simulink model "VAS_LEVEL0_TASK1_TIME"  (Simulink 3.00)
libraries: mathlib x438, logiclib x192, paramlib x18, genlib x3, timelib x1
(part 1 of 2)

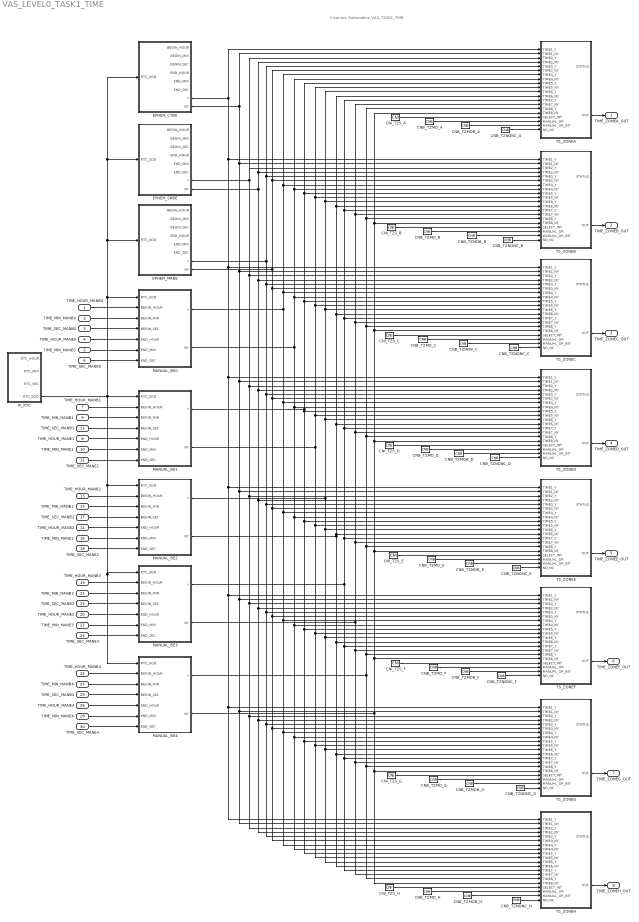
== system VAS_LEVEL0_TASK1_TIME ==
  note: Vivarium Automation VAS_TASK1_TIME
  TIME_HOUR_MANB0 : Inport  Port=1
  TIME_MIN_MANB0 : Inport  Port=2
  TIME_SEC_MANB0 : Inport  Port=3
  TIME_HOUR_MANE0 : Inport  Port=4
  TIME_MIN_MANE0 : Inport  Port=5
  TIME_SEC_MANE0 : Inport  Port=6
  TIME_HOUR_MANB1 : Inport  Port=7
  TIME_HOUR_MANE1 : Inport  Port=8
  TIME_MIN_MANB1 : Inport  Port=9
  TIME_MIN_MANE1 : Inport  Port=10
  TIME_SEC_MANB1 : Inport  Port=11
  TIME_SEC_MANE1 : Inport  Port=12
  TIME_HOUR_MANB2 : Inport  Port=13
  TIME_HOUR_MANE2 : Inport  Port=14
  TIME_MIN_MANB2 : Inport  Port=15
  TIME_MIN_MANE2 : Inport  Port=16
  TIME_SEC_MANB2 : Inport  Port=17
  TIME_SEC_MANE2 : Inport  Port=18
  TIME_HOUR_MANB3 : Inport  Port=19
  TIME_HOUR_MANE3 : Inport  Port=20
  TIME_MIN_MANB3 : Inport  Port=21
  TIME_MIN_MANE3 : Inport  Port=22
  TIME_SEC_MANB3 : Inport  Port=23
  TIME_SEC_MANE3 : Inport  Port=24
  TIME_HOUR_MANB4 : Inport  Port=25
  TIME_HOUR_MANE4 : Inport  Port=26
  TIME_MIN_MANB4 : Inport  Port=27
  TIME_MIN_MANE4 : Inport  Port=28
  TIME_SEC_MANB4 : Inport  Port=29
  TIME_SEC_MANE4 : Inport  Port=30
  CNB_TZMOB_A : mathlib/CNB  YCN=off
  CNB_TZMOB_B : mathlib/CNB  YCN=off
  CNB_TZMOB_C : mathlib/CNB  YCN=off
  CNB_TZMOB_D : mathlib/CNB  YCN=off
  CNB_TZMOB_E : mathlib/CNB  YCN=off
  CNB_TZMOB_F : mathlib/CNB  YCN=off
  CNB_TZMOB_G : mathlib/CNB  YCN=off
  CNB_TZMOB_H : mathlib/CNB  YCN=off
  CNB_TZMO_A : mathlib/CNB  YCN=off
  CNB_TZMO_B : mathlib/CNB  YCN=off
  CNB_TZMO_C : mathlib/CNB  YCN=off
  CNB_TZMO_D : mathlib/CNB  YCN=off
  CNB_TZMO_E : mathlib/CNB  YCN=off
  CNB_TZMO_F : mathlib/CNB  YCN=off
  CNB_TZMO_G : mathlib/CNB  YCN=off
  CNB_TZMO_H : mathlib/CNB  YCN=off
  CNB_TZNONC_A : mathlib/CNB  YCN=on
  CNB_TZNONC_B : mathlib/CNB  YCN=on
  CNB_TZNONC_C : mathlib/CNB  YCN=on
  CNB_TZNONC_D : mathlib/CNB  YCN=on
  CNB_TZNONC_E : mathlib/CNB  YCN=off
  CNB_TZNONC_F : mathlib/CNB  YCN=off
  CNB_TZNONC_G : mathlib/CNB  YCN=off
  CNB_TZNONC_H : mathlib/CNB  YCN=off
  CNI_TZS_A : mathlib/CNI  icn=0
  CNI_TZS_B : mathlib/CNI  icn=2
  CNI_TZS_C : mathlib/CNI  icn=1
  CNI_TZS_D : mathlib/CNI  icn=6
  CNI_TZS_E : mathlib/CNI  icn=16
  CNI_TZS_F : mathlib/CNI  icn=16
  CNI_TZS_G : mathlib/CNI  icn=16
  CNI_TZS_H : mathlib/CNI  icn=16
  EPHEM_CTBE : Subsystem
      mask Type: REX sequence
  EPHEM_MRBE : Subsystem
      mask Type: REX sequence
  EPHEM_SRBE : Subsystem
      mask Type: REX sequence
  MANUAL_BE0 : Subsystem
      mask Type: REX sequence
  MANUAL_BE1 : Subsystem
      mask Type: REX sequence
  MANUAL_BE2 : Subsystem
      mask Type: REX sequence
  MANUAL_BE3 : Subsystem
      mask Type: REX sequence
  MANUAL_BE4 : Subsystem
      mask Type: REX sequence
  PI_RTC : Subsystem
      mask Type: REX sequence
  TS_ZONEA : Subsystem
      mask Type: REX sequence
  TS_ZONEB : Subsystem
      mask Type: REX sequence
  TS_ZONEC : Subsystem
      mask Type: REX sequence
  TS_ZONED : Subsystem
      mask Type: REX sequence
  TS_ZONEE : Subsystem
      mask Type: REX sequence
  TS_ZONEF : Subsystem
      mask Type: REX sequence
  TS_ZONEG : Subsystem
      mask Type: REX sequence
  TS_ZONEH : Subsystem
      mask Type: REX sequence
  TIME_ZONEA_OUT : Outport  Port=1
  TIME_ZONEB_OUT : Outport  Port=2
  TIME_ZONEC_OUT : Outport  Port=3
  TIME_ZONED_OUT : Outport  Port=4
  TIME_ZONEE_OUT : Outport  Port=5
  TIME_ZONEF_OUT : Outport  Port=6
  TIME_ZONEG_OUT : Outport  Port=7
  TIME_ZONEH_OUT : Outport  Port=8
  wires:
  CNB_TZMOB_A/1 -> TS_ZONEA/19(MANUAL_OR_BIT)
  CNB_TZMOB_B/1 -> TS_ZONEB/19(MANUAL_OR_BIT)
  CNB_TZMOB_C/1 -> TS_ZONEC/19(MANUAL_OR_BIT)
  CNB_TZMOB_D/1 -> TS_ZONED/19(MANUAL_OR_BIT)
  CNB_TZMOB_E/1 -> TS_ZONEE/19(MANUAL_OR_BIT)
  CNB_TZMOB_F/1 -> TS_ZONEF/19(MANUAL_OR_BIT)
  CNB_TZMOB_G/1 -> TS_ZONEG/19(MANUAL_OR_BIT)
  CNB_TZMOB_H/1 -> TS_ZONEH/19(MANUAL_OR_BIT)
  CNB_TZMO_A/1 -> TS_ZONEA/18(MANUAL_OR)
  CNB_TZMO_B/1 -> TS_ZONEB/18(MANUAL_OR)
  CNB_TZMO_C/1 -> TS_ZONEC/18(MANUAL_OR)
  CNB_TZMO_D/1 -> TS_ZONED/18(MANUAL_OR)
  CNB_TZMO_E/1 -> TS_ZONEE/18(MANUAL_OR)
  CNB_TZMO_F/1 -> TS_ZONEF/18(MANUAL_OR)
  CNB_TZMO_G/1 -> TS_ZONEG/18(MANUAL_OR)
  CNB_TZMO_H/1 -> TS_ZONEH/18(MANUAL_OR)
  CNB_TZNONC_A/1 -> TS_ZONEA/20(NO_NC)
  CNB_TZNONC_B/1 -> TS_ZONEB/20(NO_NC)
  CNB_TZNONC_C/1 -> TS_ZONEC/20(NO_NC)
  CNB_TZNONC_D/1 -> TS_ZONED/20(NO_NC)
  CNB_TZNONC_E/1 -> TS_ZONEE/20(NO_NC)
  CNB_TZNONC_F/1 -> TS_ZONEF/20(NO_NC)
  CNB_TZNONC_G/1 -> TS_ZONEG/20(NO_NC)
  CNB_TZNONC_H/1 -> TS_ZONEH/20(NO_NC)
  CNI_TZS_A/1 -> TS_ZONEA/17(SELECT_INT)
  CNI_TZS_B/1 -> TS_ZONEB/17(SELECT_INT)
  CNI_TZS_C/1 -> TS_ZONEC/17(SELECT_INT)
  CNI_TZS_D/1 -> TS_ZONED/17(SELECT_INT)
  CNI_TZS_E/1 -> TS_ZONEE/17(SELECT_INT)
  CNI_TZS_F/1 -> TS_ZONEF/17(SELECT_INT)
  CNI_TZS_G/1 -> TS_ZONEG/17(SELECT_INT)
  CNI_TZS_H/1 -> TS_ZONEH/17(SELECT_INT)
  EPHEM_CTBE/7(Y) -> TS_ZONEA/1(TIME1_Y), TS_ZONEB/1(TIME1_Y), TS_ZONEC/1(TIME1_Y), TS_ZONED/1(TIME1_Y), TS_ZONEE/1(TIME1_Y), TS_ZONEG/1(TIME1_Y), TS_ZONEH/1(TIME1_Y), TS_ZONEF/1(TIME1_Y)
  EPHEM_CTBE/8(NY) -> TS_ZONEA/2(TIME1_NY), TS_ZONEB/2(TIME1_NY), TS_ZONEC/2(TIME1_NY), TS_ZONED/2(TIME1_NY), TS_ZONEE/2(TIME1_NY), TS_ZONEG/2(TIME1_NY), TS_ZONEH/2(TIME1_NY), TS_ZONEF/2(TIME1_NY)
  EPHEM_MRBE/7(Y) -> TS_ZONEA/5(TIME3_Y), TS_ZONEB/5(TIME3_Y), TS_ZONEC/5(TIME3_Y), TS_ZONED/5(TIME3_Y), TS_ZONEE/5(TIME3_Y), TS_ZONEG/5(TIME3_Y), TS_ZONEH/5(TIME3_Y), TS_ZONEF/5(TIME3_Y)
  EPHEM_MRBE/8(NY) -> TS_ZONEA/6(TIME3_NY), TS_ZONEB/6(TIME3_NY), TS_ZONEC/6(TIME3_NY), TS_ZONED/6(TIME3_NY), TS_ZONEE/6(TIME3_NY), TS_ZONEG/6(TIME3_NY), TS_ZONEH/6(TIME3_NY), TS_ZONEF/6(TIME3_NY)
  EPHEM_SRBE/7(Y) -> TS_ZONEC/3(TIME2_Y), TS_ZONED/3(TIME2_Y), TS_ZONEE/3(TIME2_Y), TS_ZONEG/3(TIME2_Y), TS_ZONEH/3(TIME2_Y), TS_ZONEF/3(TIME2_Y), TS_ZONEA/3(TIME2_Y), TS_ZONEB/3(TIME2_Y)
  EPHEM_SRBE/8(NY) -> TS_ZONEA/4(TIME2_NY), TS_ZONEB/4(TIME2_NY), TS_ZONEC/4(TIME2_NY), TS_ZONED/4(TIME2_NY), TS_ZONEE/4(TIME2_NY), TS_ZONEG/4(TIME2_NY), TS_ZONEH/4(TIME2_NY), TS_ZONEF/4(TIME2_NY)
  MANUAL_BE0/1(Y) -> TS_ZONEA/7(TIME4_Y), TS_ZONEB/7(TIME4_Y), TS_ZONEC/7(TIME4_Y), TS_ZONED/7(TIME4_Y), TS_ZONEE/7(TIME4_Y), TS_ZONEG/7(TIME4_Y), TS_ZONEH/7(TIME4_Y), TS_ZONEF/7(TIME4_Y)
  MANUAL_BE0/2(NY) -> TS_ZONEA/8(TIME4_NY), TS_ZONEB/8(TIME4_NY), TS_ZONEC/8(TIME4_NY), TS_ZONED/8(TIME4_NY), TS_ZONEE/8(TIME4_NY), TS_ZONEG/8(TIME4_NY), TS_ZONEH/8(TIME4_NY), TS_ZONEF/8(TIME4_NY)
  MANUAL_BE1/1(Y) -> TS_ZONEA/9(TIME5_Y), TS_ZONEB/9(TIME5_Y), TS_ZONEC/9(TIME5_Y), TS_ZONED/9(TIME5_Y), TS_ZONEE/9(TIME5_Y), TS_ZONEG/9(TIME5_Y), TS_ZONEH/9(TIME5_Y), TS_ZONEF/9(TIME5_Y)
  MANUAL_BE1/2(NY) -> TS_ZONEA/10(TIME5_NY), TS_ZONEB/10(TIME5_NY), TS_ZONEC/10(TIME5_NY), TS_ZONED/10(TIME5_NY), TS_ZONEE/10(TIME5_NY), TS_ZONEG/10(TIME5_NY), TS_ZONEH/10(TIME5_NY), TS_ZONEF/10(TIME5_NY)
  MANUAL_BE2/1(Y) -> TS_ZONEA/11(TIME6_Y), TS_ZONEB/11(TIME6_Y), TS_ZONEC/11(TIME6_Y), TS_ZONED/11(TIME6_Y), TS_ZONEE/11(TIME6_Y), TS_ZONEG/11(TIME6_Y), TS_ZONEH/11(TIME6_Y), TS_ZONEF/11(TIME6_Y)
  MANUAL_BE2/2(NY) -> TS_ZONEA/12(TIME6_NY), TS_ZONEB/12(TIME6_NY), TS_ZONEC/12(TIME6_NY), TS_ZONED/12(TIME6_NY), TS_ZONEE/12(TIME6_NY), TS_ZONEG/12(TIME6_NY), TS_ZONEH/12(TIME6_NY), TS_ZONEF/12(TIME6_NY)
  MANUAL_BE3/1(Y) -> TS_ZONEA/13(TIME7_Y), TS_ZONEB/13(TIME7_Y), TS_ZONEC/13(TIME7_Y), TS_ZONED/13(TIME7_Y), TS_ZONEE/13(TIME7_Y), TS_ZONEG/13(TIME7_Y), TS_ZONEH/13(TIME7_Y), TS_ZONEF/13(TIME7_Y)
  MANUAL_BE3/2(NY) -> TS_ZONEA/14(TIME7_NY), TS_ZONEB/14(TIME7_NY), TS_ZONEC/14(TIME7_NY), TS_ZONED/14(TIME7_NY), TS_ZONEE/14(TIME7_NY), TS_ZONEG/14(TIME7_NY), TS_ZONEH/14(TIME7_NY), TS_ZONEF/14(TIME7_NY)
  MANUAL_BE4/1(Y) -> TS_ZONEA/15(TIME8_Y), TS_ZONEB/15(TIME8_Y), TS_ZONEC/15(TIME8_Y), TS_ZONED/15(TIME8_Y), TS_ZONEE/15(TIME8_Y), TS_ZONEF/15(TIME8_Y), TS_ZONEG/15(TIME8_Y), TS_ZONEH/15(TIME8_Y)
  MANUAL_BE4/2(NY) -> TS_ZONEA/16(TIME8_NY), TS_ZONEB/16(TIME8_NY), TS_ZONEC/16(TIME8_NY), TS_ZONED/16(TIME8_NY), TS_ZONEE/16(TIME8_NY), TS_ZONEF/16(TIME8_NY), TS_ZONEG/16(TIME8_NY), TS_ZONEH/16(TIME8_NY)
  PI_RTC/4(RTC_SOD) -> MANUAL_BE3/1(RTC_SOD), MANUAL_BE4/1(RTC_SOD), MANUAL_BE2/1(RTC_SOD), EPHEM_CTBE/1(RTC_SOD), EPHEM_SRBE/1(RTC_SOD), EPHEM_MRBE/1(RTC_SOD), MANUAL_BE0/1(RTC_SOD), MANUAL_BE1/1(RTC_SOD)
  TIME_HOUR_MANB0/1 -> MANUAL_BE0/2(BEGIN_HOUR)
  TIME_HOUR_MANB1/1 -> MANUAL_BE1/2(BEGIN_HOUR)
  TIME_HOUR_MANB2/1 -> MANUAL_BE2/2(BEGIN_HOUR)
  TIME_HOUR_MANB3/1 -> MANUAL_BE3/2(BEGIN_HOUR)
  TIME_HOUR_MANB4/1 -> MANUAL_BE4/2(BEGIN_HOUR)
  TIME_HOUR_MANE0/1 -> MANUAL_BE0/5(END_HOUR)
  TIME_HOUR_MANE1/1 -> MANUAL_BE1/5(END_HOUR)
  TIME_HOUR_MANE2/1 -> MANUAL_BE2/5(END_HOUR)
  TIME_HOUR_MANE3/1 -> MANUAL_BE3/5(END_HOUR)
  TIME_HOUR_MANE4/1 -> MANUAL_BE4/5(END_HOUR)
  TIME_MIN_MANB0/1 -> MANUAL_BE0/3(BEGIN_MIN)
  TIME_MIN_MANB1/1 -> MANUAL_BE1/3(BEGIN_MIN)
  TIME_MIN_MANB2/1 -> MANUAL_BE2/3(BEGIN_MIN)
  TIME_MIN_MANB3/1 -> MANUAL_BE3/3(BEGIN_MIN)
  TIME_MIN_MANB4/1 -> MANUAL_BE4/3(BEGIN_MIN)
  TIME_MIN_MANE0/1 -> MANUAL_BE0/6(END_MIN)
  TIME_MIN_MANE1/1 -> MANUAL_BE1/6(END_MIN)
  TIME_MIN_MANE2/1 -> MANUAL_BE2/6(END_MIN)
  TIME_MIN_MANE3/1 -> MANUAL_BE3/6(END_MIN)
  TIME_MIN_MANE4/1 -> MANUAL_BE4/6(END_MIN)
  TIME_SEC_MANB0/1 -> MANUAL_BE0/4(BEGIN_SEC)
  TIME_SEC_MANB1/1 -> MANUAL_BE1/4(BEGIN_SEC)
  TIME_SEC_MANB2/1 -> MANUAL_BE2/4(BEGIN_SEC)
  TIME_SEC_MANB3/1 -> MANUAL_BE3/4(BEGIN_SEC)
  TIME_SEC_MANB4/1 -> MANUAL_BE4/4(BEGIN_SEC)
  TIME_SEC_MANE0/1 -> MANUAL_BE0/7(END_SEC)
  TIME_SEC_MANE1/1 -> MANUAL_BE1/7(END_SEC)
  TIME_SEC_MANE2/1 -> MANUAL_BE2/7(END_SEC)
  TIME_SEC_MANE3/1 -> MANUAL_BE3/7(END_SEC)
  TIME_SEC_MANE4/1 -> MANUAL_BE4/7(END_SEC)
  TS_ZONEA/2(OUT) -> TIME_ZONEA_OUT/1
  TS_ZONEB/2(OUT) -> TIME_ZONEB_OUT/1
  TS_ZONEC/2(OUT) -> TIME_ZONEC_OUT/1
  TS_ZONED/2(OUT) -> TIME_ZONED_OUT/1
  TS_ZONEE/2(OUT) -> TIME_ZONEE_OUT/1
  TS_ZONEF/2(OUT) -> TIME_ZONEF_OUT/1
  TS_ZONEG/2(OUT) -> TIME_ZONEG_OUT/1
  TS_ZONEH/2(OUT) -> TIME_ZONEH_OUT/1

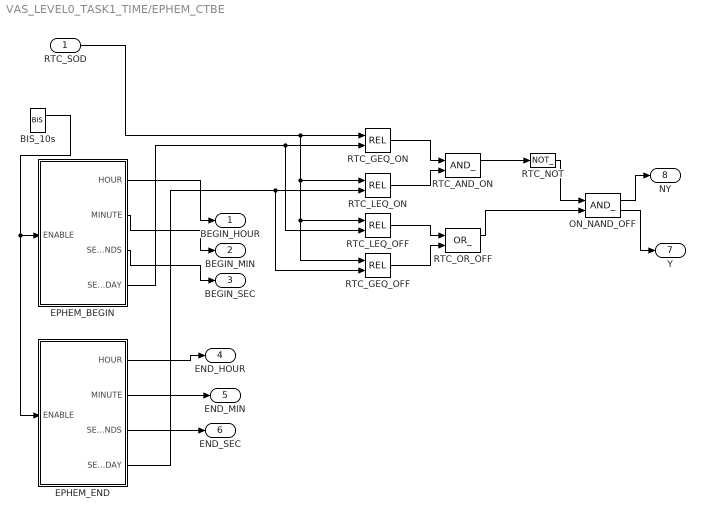
== system VAS_LEVEL0_TASK1_TIME/EPHEM_CTBE ==
  RTC_SOD : Inport  Port=1
  BIS_10s : genlib/BIS  Y0=off  t1=0  t2=1  t3=30  t4=4  t5=5  t6=6  t7=7  t8=8  RPT=on  bEdit=off
  EPHEM_BEGIN : Subsystem
      mask Type: REX sequence
  EPHEM_END : Subsystem
      mask Type: REX sequence
  ON_NAND_OFF : logiclib/AND_
  RTC_AND_ON : logiclib/AND_
  RTC_GEQ_OFF : mathlib/REL  irel=6: greater or equal (>=)
  RTC_GEQ_ON : mathlib/REL  irel=6: greater or equal (>=)
  RTC_LEQ_OFF : mathlib/REL  irel=5: less or equal (<=)
  RTC_LEQ_ON : mathlib/REL  irel=5: less or equal (<=)
  RTC_NOT : logiclib/NOT_
  RTC_OR_OFF : logiclib/OR_
  BEGIN_HOUR : Outport  Port=1
  BEGIN_MIN : Outport  Port=2
  BEGIN_SEC : Outport  Port=3
  END_HOUR : Outport  Port=4
  END_MIN : Outport  Port=5
  END_SEC : Outport  Port=6
  Y : Outport  Port=7
  NY : Outport  Port=8
  wires:
  BIS_10s/1 -> EPHEM_BEGIN/1(ENABLE), EPHEM_END/1(ENABLE)
  EPHEM_BEGIN/1(HOUR) -> BEGIN_HOUR/1
  EPHEM_BEGIN/2(MINUTE) -> BEGIN_MIN/1
  EPHEM_BEGIN/3(SECONDS) -> BEGIN_SEC/1
  EPHEM_BEGIN/4(SEC_OF_DAY) -> RTC_GEQ_ON/2, RTC_LEQ_OFF/2
  EPHEM_END/1(HOUR) -> END_HOUR/1
  EPHEM_END/2(MINUTE) -> END_MIN/1
  EPHEM_END/3(SECONDS) -> END_SEC/1
  EPHEM_END/4(SEC_OF_DAY) -> RTC_GEQ_OFF/2, RTC_LEQ_ON/2
  ON_NAND_OFF/1 -> NY/1
  ON_NAND_OFF/2 -> Y/1
  RTC_AND_ON/1 -> RTC_NOT/1
  RTC_GEQ_OFF/1 -> RTC_OR_OFF/2
  RTC_GEQ_ON/1 -> RTC_AND_ON/1
  RTC_LEQ_OFF/1 -> RTC_OR_OFF/1
  RTC_LEQ_ON/1 -> RTC_AND_ON/2
  RTC_NOT/1 -> ON_NAND_OFF/1
  RTC_OR_OFF/1 -> ON_NAND_OFF/2
  RTC_SOD/1 -> RTC_GEQ_ON/1, RTC_GEQ_OFF/1, RTC_LEQ_OFF/1, RTC_LEQ_ON/1

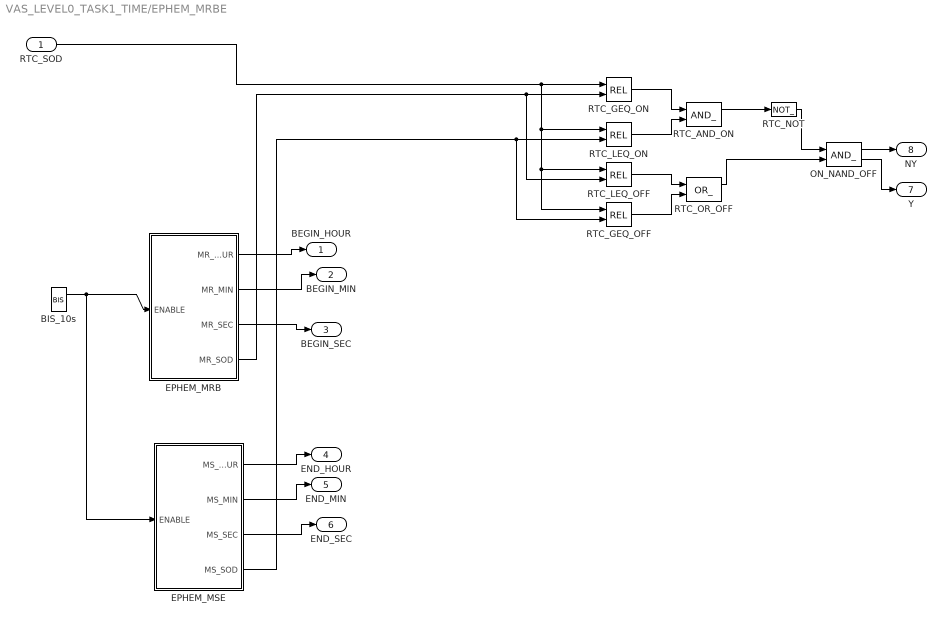
== system VAS_LEVEL0_TASK1_TIME/EPHEM_MRBE ==
  RTC_SOD : Inport  Port=1
  BIS_10s : genlib/BIS  Y0=off  t1=0  t2=1  t3=30  t4=4  t5=5  t6=6  t7=7  t8=8  RPT=on  bEdit=off
  EPHEM_MRB : Subsystem
      mask Type: REX sequence
  EPHEM_MSE : Subsystem
      mask Type: REX sequence
  ON_NAND_OFF : logiclib/AND_
  RTC_AND_ON : logiclib/AND_
  RTC_GEQ_OFF : mathlib/REL  irel=6: greater or equal (>=)
  RTC_GEQ_ON : mathlib/REL  irel=6: greater or equal (>=)
  RTC_LEQ_OFF : mathlib/REL  irel=5: less or equal (<=)
  RTC_LEQ_ON : mathlib/REL  irel=5: less or equal (<=)
  RTC_NOT : logiclib/NOT_
  RTC_OR_OFF : logiclib/OR_
  BEGIN_HOUR : Outport  Port=1
  BEGIN_MIN : Outport  Port=2
  BEGIN_SEC : Outport  Port=3
  END_HOUR : Outport  Port=4
  END_MIN : Outport  Port=5
  END_SEC : Outport  Port=6
  Y : Outport  Port=7
  NY : Outport  Port=8
  wires:
  BIS_10s/1 -> EPHEM_MRB/1(ENABLE), EPHEM_MSE/1(ENABLE)
  EPHEM_MRB/1(MR_HOUR) -> BEGIN_HOUR/1
  EPHEM_MRB/2(MR_MIN) -> BEGIN_MIN/1
  EPHEM_MRB/3(MR_SEC) -> BEGIN_SEC/1
  EPHEM_MRB/4(MR_SOD) -> RTC_GEQ_ON/2, RTC_LEQ_OFF/2
  EPHEM_MSE/1(MS_HOUR) -> END_HOUR/1
  EPHEM_MSE/2(MS_MIN) -> END_MIN/1
  EPHEM_MSE/3(MS_SEC) -> END_SEC/1
  EPHEM_MSE/4(MS_SOD) -> RTC_GEQ_OFF/2, RTC_LEQ_ON/2
  ON_NAND_OFF/1 -> NY/1
  ON_NAND_OFF/2 -> Y/1
  RTC_AND_ON/1 -> RTC_NOT/1
  RTC_GEQ_OFF/1 -> RTC_OR_OFF/2
  RTC_GEQ_ON/1 -> RTC_AND_ON/1
  RTC_LEQ_OFF/1 -> RTC_OR_OFF/1
  RTC_LEQ_ON/1 -> RTC_AND_ON/2
  RTC_NOT/1 -> ON_NAND_OFF/1
  RTC_OR_OFF/1 -> ON_NAND_OFF/2
  RTC_SOD/1 -> RTC_GEQ_ON/1, RTC_GEQ_OFF/1, RTC_LEQ_OFF/1, RTC_LEQ_ON/1

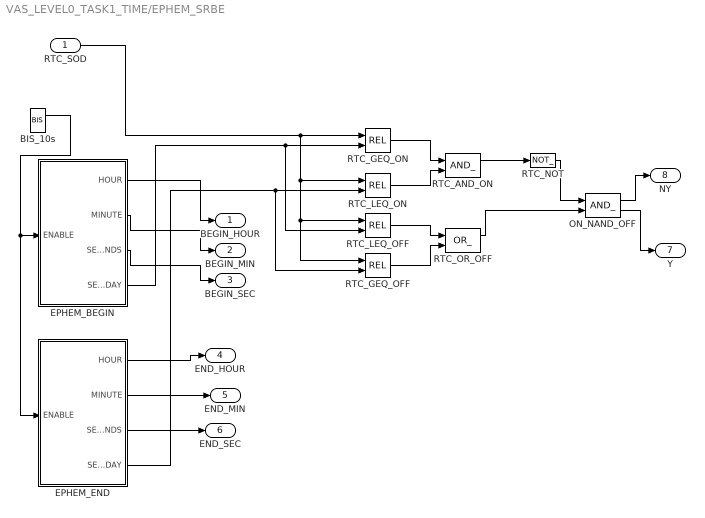
== system VAS_LEVEL0_TASK1_TIME/EPHEM_SRBE ==
  RTC_SOD : Inport  Port=1
  BIS_10s : genlib/BIS  Y0=off  t1=0  t2=1  t3=30  t4=4  t5=5  t6=6  t7=7  t8=8  RPT=on  bEdit=off
  EPHEM_BEGIN : Subsystem
      mask Type: REX sequence
  EPHEM_END : Subsystem
      mask Type: REX sequence
  ON_NAND_OFF : logiclib/AND_
  RTC_AND_ON : logiclib/AND_
  RTC_GEQ_OFF : mathlib/REL  irel=6: greater or equal (>=)
  RTC_GEQ_ON : mathlib/REL  irel=6: greater or equal (>=)
  RTC_LEQ_OFF : mathlib/REL  irel=5: less or equal (<=)
  RTC_LEQ_ON : mathlib/REL  irel=5: less or equal (<=)
  RTC_NOT : logiclib/NOT_
  RTC_OR_OFF : logiclib/OR_
  BEGIN_HOUR : Outport  Port=1
  BEGIN_MIN : Outport  Port=2
  BEGIN_SEC : Outport  Port=3
  END_HOUR : Outport  Port=4
  END_MIN : Outport  Port=5
  END_SEC : Outport  Port=6
  Y : Outport  Port=7
  NY : Outport  Port=8
  wires:
  BIS_10s/1 -> EPHEM_BEGIN/1(ENABLE), EPHEM_END/1(ENABLE)
  EPHEM_BEGIN/1(HOUR) -> BEGIN_HOUR/1
  EPHEM_BEGIN/2(MINUTE) -> BEGIN_MIN/1
  EPHEM_BEGIN/3(SECONDS) -> BEGIN_SEC/1
  EPHEM_BEGIN/4(SEC_OF_DAY) -> RTC_GEQ_ON/2, RTC_LEQ_OFF/2
  EPHEM_END/1(HOUR) -> END_HOUR/1
  EPHEM_END/2(MINUTE) -> END_MIN/1
  EPHEM_END/3(SECONDS) -> END_SEC/1
  EPHEM_END/4(SEC_OF_DAY) -> RTC_GEQ_OFF/2, RTC_LEQ_ON/2
  ON_NAND_OFF/1 -> NY/1
  ON_NAND_OFF/2 -> Y/1
  RTC_AND_ON/1 -> RTC_NOT/1
  RTC_GEQ_OFF/1 -> RTC_OR_OFF/2
  RTC_GEQ_ON/1 -> RTC_AND_ON/1
  RTC_LEQ_OFF/1 -> RTC_OR_OFF/1
  RTC_LEQ_ON/1 -> RTC_AND_ON/2
  RTC_NOT/1 -> ON_NAND_OFF/1
  RTC_OR_OFF/1 -> ON_NAND_OFF/2
  RTC_SOD/1 -> RTC_GEQ_ON/1, RTC_GEQ_OFF/1, RTC_LEQ_OFF/1, RTC_LEQ_ON/1

== system VAS_LEVEL0_TASK1_TIME/MANUAL_BE0 ==
  RTC_SOD : Inport  Port=1
  BEGIN_HOUR : Inport  Port=2
  BEGIN_MIN : Inport  Port=3
  BEGIN_SEC : Inport  Port=4
  END_HOUR : Inport  Port=5
  END_MIN : Inport  Port=6
  END_SEC : Inport  Port=7
  MANUAL_BEGIN : Subsystem
      mask Type: REX sequence
  MANUAL_END : Subsystem
      mask Type: REX sequence
  ON_NAND_OFF : logiclib/AND_
  RTC_AND_ON : logiclib/AND_
  RTC_GEQ_OFF : mathlib/REL  irel=6: greater or equal (>=)
  RTC_GEQ_ON : mathlib/REL  irel=6: greater or equal (>=)
  RTC_LEQ_OFF : mathlib/REL  irel=5: less or equal (<=)
  RTC_LEQ_ON : mathlib/REL  irel=5: less or equal (<=)
  RTC_NOT : logiclib/NOT_
  RTC_OR_OFF : logiclib/OR_
  Y : Outport  Port=1
  NY : Outport  Port=2
  wires:
  BEGIN_HOUR/1 -> MANUAL_BEGIN/1(IN_HOUR)
  BEGIN_MIN/1 -> MANUAL_BEGIN/2(IN_MINUTE)
  BEGIN_SEC/1 -> MANUAL_BEGIN/3(IN_SECONDS)
  END_HOUR/1 -> MANUAL_END/1(IN_HOUR)
  END_MIN/1 -> MANUAL_END/2(IN_MINUTE)
  END_SEC/1 -> MANUAL_END/3(IN_SECONDS)
  MANUAL_BEGIN/4(SEC_OF_DAY) -> RTC_GEQ_ON/2, RTC_LEQ_OFF/2
  MANUAL_END/4(SEC_OF_DAY) -> RTC_GEQ_OFF/2, RTC_LEQ_ON/2
  ON_NAND_OFF/1 -> NY/1
  ON_NAND_OFF/2 -> Y/1
  RTC_AND_ON/1 -> RTC_NOT/1
  RTC_GEQ_OFF/1 -> RTC_OR_OFF/2
  RTC_GEQ_ON/1 -> RTC_AND_ON/1
  RTC_LEQ_OFF/1 -> RTC_OR_OFF/1
  RTC_LEQ_ON/1 -> RTC_AND_ON/2
  RTC_NOT/1 -> ON_NAND_OFF/1
  RTC_OR_OFF/1 -> ON_NAND_OFF/2
  RTC_SOD/1 -> RTC_GEQ_ON/1, RTC_GEQ_OFF/1, RTC_LEQ_OFF/1, RTC_LEQ_ON/1

== system VAS_LEVEL0_TASK1_TIME/MANUAL_BE1 ==
  RTC_SOD : Inport  Port=1
  BEGIN_HOUR : Inport  Port=2
  BEGIN_MIN : Inport  Port=3
  BEGIN_SEC : Inport  Port=4
  END_HOUR : Inport  Port=5
  END_MIN : Inport  Port=6
  END_SEC : Inport  Port=7
  MANUAL_BEGIN : Subsystem
      mask Type: REX sequence
  MANUAL_END : Subsystem
      mask Type: REX sequence
  ON_NAND_OFF : logiclib/AND_
  RTC_AND_ON : logiclib/AND_
  RTC_GEQ_OFF : mathlib/REL  irel=6: greater or equal (>=)
  RTC_GEQ_ON : mathlib/REL  irel=6: greater or equal (>=)
  RTC_LEQ_OFF : mathlib/REL  irel=5: less or equal (<=)
  RTC_LEQ_ON : mathlib/REL  irel=5: less or equal (<=)
  RTC_NOT : logiclib/NOT_
  RTC_OR_OFF : logiclib/OR_
  Y : Outport  Port=1
  NY : Outport  Port=2
  wires:
  BEGIN_HOUR/1 -> MANUAL_BEGIN/1(IN_HOUR)
  BEGIN_MIN/1 -> MANUAL_BEGIN/2(IN_MINUTE)
  BEGIN_SEC/1 -> MANUAL_BEGIN/3(IN_SECONDS)
  END_HOUR/1 -> MANUAL_END/1(IN_HOUR)
  END_MIN/1 -> MANUAL_END/2(IN_MINUTE)
  END_SEC/1 -> MANUAL_END/3(IN_SECONDS)
  MANUAL_BEGIN/4(SEC_OF_DAY) -> RTC_GEQ_ON/2, RTC_LEQ_OFF/2
  MANUAL_END/4(SEC_OF_DAY) -> RTC_GEQ_OFF/2, RTC_LEQ_ON/2
  ON_NAND_OFF/1 -> NY/1
  ON_NAND_OFF/2 -> Y/1
  RTC_AND_ON/1 -> RTC_NOT/1
  RTC_GEQ_OFF/1 -> RTC_OR_OFF/2
  RTC_GEQ_ON/1 -> RTC_AND_ON/1
  RTC_LEQ_OFF/1 -> RTC_OR_OFF/1
  RTC_LEQ_ON/1 -> RTC_AND_ON/2
  RTC_NOT/1 -> ON_NAND_OFF/1
  RTC_OR_OFF/1 -> ON_NAND_OFF/2
  RTC_SOD/1 -> RTC_GEQ_ON/1, RTC_GEQ_OFF/1, RTC_LEQ_OFF/1, RTC_LEQ_ON/1

== system VAS_LEVEL0_TASK1_TIME/MANUAL_BE2 ==
  RTC_SOD : Inport  Port=1
  BEGIN_HOUR : Inport  Port=2
  BEGIN_MIN : Inport  Port=3
  BEGIN_SEC : Inport  Port=4
  END_HOUR : Inport  Port=5
  END_MIN : Inport  Port=6
  END_SEC : Inport  Port=7
  MANUAL_BEGIN : Subsystem
      mask Type: REX sequence
  MANUAL_END : Subsystem
      mask Type: REX sequence
  ON_NAND_OFF : logiclib/AND_
  RTC_AND_ON : logiclib/AND_
  RTC_GEQ_OFF : mathlib/REL  irel=6: greater or equal (>=)
  RTC_GEQ_ON : mathlib/REL  irel=6: greater or equal (>=)
  RTC_LEQ_OFF : mathlib/REL  irel=5: less or equal (<=)
  RTC_LEQ_ON : mathlib/REL  irel=5: less or equal (<=)
  RTC_NOT : logiclib/NOT_
  RTC_OR_OFF : logiclib/OR_
  Y : Outport  Port=1
  NY : Outport  Port=2
  wires:
  BEGIN_HOUR/1 -> MANUAL_BEGIN/1(IN_HOUR)
  BEGIN_MIN/1 -> MANUAL_BEGIN/2(IN_MINUTE)
  BEGIN_SEC/1 -> MANUAL_BEGIN/3(IN_SECONDS)
  END_HOUR/1 -> MANUAL_END/1(IN_HOUR)
  END_MIN/1 -> MANUAL_END/2(IN_MINUTE)
  END_SEC/1 -> MANUAL_END/3(IN_SECONDS)
  MANUAL_BEGIN/4(SEC_OF_DAY) -> RTC_GEQ_ON/2, RTC_LEQ_OFF/2
  MANUAL_END/4(SEC_OF_DAY) -> RTC_GEQ_OFF/2, RTC_LEQ_ON/2
  ON_NAND_OFF/1 -> NY/1
  ON_NAND_OFF/2 -> Y/1
  RTC_AND_ON/1 -> RTC_NOT/1
  RTC_GEQ_OFF/1 -> RTC_OR_OFF/2
  RTC_GEQ_ON/1 -> RTC_AND_ON/1
  RTC_LEQ_OFF/1 -> RTC_OR_OFF/1
  RTC_LEQ_ON/1 -> RTC_AND_ON/2
  RTC_NOT/1 -> ON_NAND_OFF/1
  RTC_OR_OFF/1 -> ON_NAND_OFF/2
  RTC_SOD/1 -> RTC_GEQ_ON/1, RTC_GEQ_OFF/1, RTC_LEQ_OFF/1, RTC_LEQ_ON/1

== system VAS_LEVEL0_TASK1_TIME/MANUAL_BE3 ==
  RTC_SOD : Inport  Port=1
  BEGIN_HOUR : Inport  Port=2
  BEGIN_MIN : Inport  Port=3
  BEGIN_SEC : Inport  Port=4
  END_HOUR : Inport  Port=5
  END_MIN : Inport  Port=6
  END_SEC : Inport  Port=7
  MANUAL_BEGIN : Subsystem
      mask Type: REX sequence
  MANUAL_END : Subsystem
      mask Type: REX sequence
  ON_NAND_OFF : logiclib/AND_
  RTC_AND_ON : logiclib/AND_
  RTC_GEQ_OFF : mathlib/REL  irel=6: greater or equal (>=)
  RTC_GEQ_ON : mathlib/REL  irel=6: greater or equal (>=)
  RTC_LEQ_OFF : mathlib/REL  irel=5: less or equal (<=)
  RTC_LEQ_ON : mathlib/REL  irel=5: less or equal (<=)
  RTC_NOT : logiclib/NOT_
  RTC_OR_OFF : logiclib/OR_
  Y : Outport  Port=1
  NY : Outport  Port=2
  wires:
  BEGIN_HOUR/1 -> MANUAL_BEGIN/1(IN_HOUR)
  BEGIN_MIN/1 -> MANUAL_BEGIN/2(IN_MINUTE)
  BEGIN_SEC/1 -> MANUAL_BEGIN/3(IN_SECONDS)
  END_HOUR/1 -> MANUAL_END/1(IN_HOUR)
  END_MIN/1 -> MANUAL_END/2(IN_MINUTE)
  END_SEC/1 -> MANUAL_END/3(IN_SECONDS)
  MANUAL_BEGIN/4(SEC_OF_DAY) -> RTC_GEQ_ON/2, RTC_LEQ_OFF/2
  MANUAL_END/4(SEC_OF_DAY) -> RTC_GEQ_OFF/2, RTC_LEQ_ON/2
  ON_NAND_OFF/1 -> NY/1
  ON_NAND_OFF/2 -> Y/1
  RTC_AND_ON/1 -> RTC_NOT/1
  RTC_GEQ_OFF/1 -> RTC_OR_OFF/2
  RTC_GEQ_ON/1 -> RTC_AND_ON/1
  RTC_LEQ_OFF/1 -> RTC_OR_OFF/1
  RTC_LEQ_ON/1 -> RTC_AND_ON/2
  RTC_NOT/1 -> ON_NAND_OFF/1
  RTC_OR_OFF/1 -> ON_NAND_OFF/2
  RTC_SOD/1 -> RTC_GEQ_ON/1, RTC_GEQ_OFF/1, RTC_LEQ_OFF/1, RTC_LEQ_ON/1

== system VAS_LEVEL0_TASK1_TIME/MANUAL_BE4 ==
  RTC_SOD : Inport  Port=1
  BEGIN_HOUR : Inport  Port=2
  BEGIN_MIN : Inport  Port=3
  BEGIN_SEC : Inport  Port=4
  END_HOUR : Inport  Port=5
  END_MIN : Inport  Port=6
  END_SEC : Inport  Port=7
  MANUAL_BEGIN : Subsystem
      mask Type: REX sequence
  MANUAL_END : Subsystem
      mask Type: REX sequence
  ON_NAND_OFF : logiclib/AND_
  RTC_AND_ON : logiclib/AND_
  RTC_GEQ_OFF : mathlib/REL  irel=6: greater or equal (>=)
  RTC_GEQ_ON : mathlib/REL  irel=6: greater or equal (>=)
  RTC_LEQ_OFF : mathlib/REL  irel=5: less or equal (<=)
  RTC_LEQ_ON : mathlib/REL  irel=5: less or equal (<=)
  RTC_NOT : logiclib/NOT_
  RTC_OR_OFF : logiclib/OR_
  Y : Outport  Port=1
  NY : Outport  Port=2
  wires:
  BEGIN_HOUR/1 -> MANUAL_BEGIN/1(IN_HOUR)
  BEGIN_MIN/1 -> MANUAL_BEGIN/2(IN_MINUTE)
  BEGIN_SEC/1 -> MANUAL_BEGIN/3(IN_SECONDS)
  END_HOUR/1 -> MANUAL_END/1(IN_HOUR)
  END_MIN/1 -> MANUAL_END/2(IN_MINUTE)
  END_SEC/1 -> MANUAL_END/3(IN_SECONDS)
  MANUAL_BEGIN/4(SEC_OF_DAY) -> RTC_GEQ_ON/2, RTC_LEQ_OFF/2
  MANUAL_END/4(SEC_OF_DAY) -> RTC_GEQ_OFF/2, RTC_LEQ_ON/2
  ON_NAND_OFF/1 -> NY/1
  ON_NAND_OFF/2 -> Y/1
  RTC_AND_ON/1 -> RTC_NOT/1
  RTC_GEQ_OFF/1 -> RTC_OR_OFF/2
  RTC_GEQ_ON/1 -> RTC_AND_ON/1
  RTC_LEQ_OFF/1 -> RTC_OR_OFF/1
  RTC_LEQ_ON/1 -> RTC_AND_ON/2
  RTC_NOT/1 -> ON_NAND_OFF/1
  RTC_OR_OFF/1 -> ON_NAND_OFF/2
  RTC_SOD/1 -> RTC_GEQ_ON/1, RTC_GEQ_OFF/1, RTC_LEQ_OFF/1, RTC_LEQ_ON/1

== system VAS_LEVEL0_TASK1_TIME/PI_RTC ==
  ADD_AMS : mathlib/ADD
  ADD_HM : mathlib/ADD
  CNI_IMUL_H : mathlib/CNI  icn=3600
  CNI_IMUL_M : mathlib/CNI  icn=60
  IMUL_H : mathlib/IMUL  vtype=4: Long  SAT=off
  IMUL_M : mathlib/IMUL  vtype=4: Long  SAT=off
  PI_TIME : timelib/TIME  tz=1: Local time
  RTC_HOUR : Outport  Port=1
  RTC_MIN : Outport  Port=2
  RTC_SEC : Outport  Port=3
  RTC_SOD : Outport  Port=4
  wires:
  ADD_AMS/1 -> RTC_SOD/1
  ADD_HM/1 -> ADD_AMS/1
  CNI_IMUL_H/1 -> IMUL_H/2
  CNI_IMUL_M/1 -> IMUL_M/2
  IMUL_H/1 -> ADD_HM/1
  IMUL_M/1 -> ADD_HM/2
  PI_TIME/1 -> IMUL_H/1, RTC_HOUR/1
  PI_TIME/2 -> IMUL_M/1, RTC_MIN/1
  PI_TIME/3 -> ADD_AMS/2, RTC_SEC/1

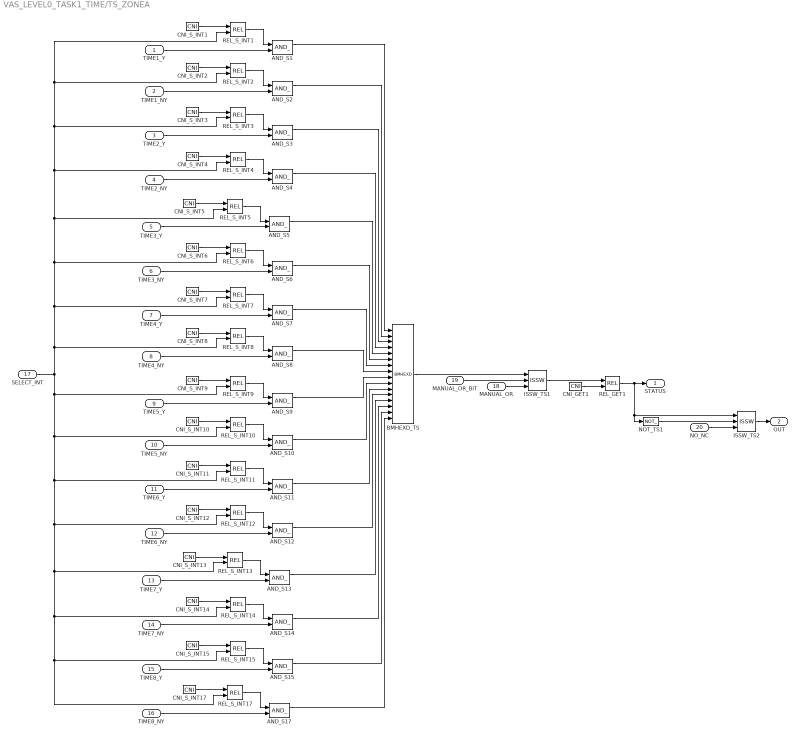
== system VAS_LEVEL0_TASK1_TIME/TS_ZONEA ==
  TIME1_Y : Inport  Port=1
  TIME1_NY : Inport  Port=2
  TIME2_Y : Inport  Port=3
  TIME2_NY : Inport  Port=4
  TIME3_Y : Inport  Port=5
  TIME3_NY : Inport  Port=6
  TIME4_Y : Inport  Port=7
  TIME4_NY : Inport  Port=8
  TIME5_Y : Inport  Port=9
  TIME5_NY : Inport  Port=10
  TIME6_Y : Inport  Port=11
  TIME6_NY : Inport  Port=12
  TIME7_Y : Inport  Port=13
  TIME7_NY : Inport  Port=14
  TIME8_Y : Inport  Port=15
  TIME8_NY : Inport  Port=16
  SELECT_INT : Inport  Port=17
  MANUAL_OR : Inport  Port=18
  MANUAL_OR_BIT : Inport  Port=19
  NO_NC : Inport  Port=20
  AND_S{1..15,17} (16 alike) : logiclib/AND_
  BMHEXD_TS : logiclib/BMHEXD  shift=0
  CNI_GET1 : mathlib/CNI  icn=1
  CNI_S_INT1 : mathlib/CNI  icn=0
  CNI_S_INT10 : mathlib/CNI  icn=9
  CNI_S_INT11 : mathlib/CNI  icn=10
  CNI_S_INT12 : mathlib/CNI  icn=11
  CNI_S_INT13 : mathlib/CNI  icn=12
  CNI_S_INT14 : mathlib/CNI  icn=13
  CNI_S_INT15 : mathlib/CNI  icn=14
  CNI_S_INT17 : mathlib/CNI  icn=15
  CNI_S_INT2 : mathlib/CNI  icn=1
  CNI_S_INT3 : mathlib/CNI  icn=2
  CNI_S_INT4 : mathlib/CNI  icn=3
  CNI_S_INT5 : mathlib/CNI  icn=4
  CNI_S_INT6 : mathlib/CNI  icn=5
  CNI_S_INT7 : mathlib/CNI  icn=6
  CNI_S_INT8 : mathlib/CNI  icn=7
  CNI_S_INT9 : mathlib/CNI  icn=8
  ISSW_TS1 : logiclib/ISSW
  ISSW_TS2 : logiclib/ISSW
  NOT_TS1 : logiclib/NOT_
  REL_GET1 : mathlib/REL  irel=6: greater or equal (>=)
  REL_S_INT{1..15,17} (16 alike) : mathlib/REL  irel=1: equality (==)
  STATUS : Outport  Port=1
  OUT : Outport  Port=2
  wires:
  AND_S1/1 -> BMHEXD_TS/1
  AND_S10/1 -> BMHEXD_TS/10
  AND_S11/1 -> BMHEXD_TS/11
  AND_S12/1 -> BMHEXD_TS/12
  AND_S13/1 -> BMHEXD_TS/13
  AND_S14/1 -> BMHEXD_TS/14
  AND_S15/1 -> BMHEXD_TS/15
  AND_S17/1 -> BMHEXD_TS/16
  AND_S2/1 -> BMHEXD_TS/2
  AND_S3/1 -> BMHEXD_TS/3
  AND_S4/1 -> BMHEXD_TS/4
  AND_S5/1 -> BMHEXD_TS/5
  AND_S6/1 -> BMHEXD_TS/6
  AND_S7/1 -> BMHEXD_TS/7
  AND_S8/1 -> BMHEXD_TS/8
  AND_S9/1 -> BMHEXD_TS/9
  BMHEXD_TS/1 -> ISSW_TS1/1
  CNI_GET1/1 -> REL_GET1/2
  CNI_S_INT1/1 -> REL_S_INT1/1
  CNI_S_INT10/1 -> REL_S_INT10/1
  CNI_S_INT11/1 -> REL_S_INT11/1
  CNI_S_INT12/1 -> REL_S_INT12/1
  CNI_S_INT13/1 -> REL_S_INT13/1
  CNI_S_INT14/1 -> REL_S_INT14/1
  CNI_S_INT15/1 -> REL_S_INT15/1
  CNI_S_INT17/1 -> REL_S_INT17/1
  CNI_S_INT2/1 -> REL_S_INT2/1
  CNI_S_INT3/1 -> REL_S_INT3/1
  CNI_S_INT4/1 -> REL_S_INT4/1
  CNI_S_INT5/1 -> REL_S_INT5/1
  CNI_S_INT6/1 -> REL_S_INT6/1
  CNI_S_INT7/1 -> REL_S_INT7/1
  CNI_S_INT8/1 -> REL_S_INT8/1
  CNI_S_INT9/1 -> REL_S_INT9/1
  ISSW_TS1/1 -> REL_GET1/1
  ISSW_TS2/1 -> OUT/1
  MANUAL_OR/1 -> ISSW_TS1/3
  MANUAL_OR_BIT/1 -> ISSW_TS1/2
  NOT_TS1/1 -> ISSW_TS2/2
  NO_NC/1 -> ISSW_TS2/3
  REL_GET1/1 -> STATUS/1, ISSW_TS2/1, NOT_TS1/1
  REL_S_INT1/1 -> AND_S1/1
  REL_S_INT10/1 -> AND_S10/1
  REL_S_INT11/1 -> AND_S11/1
  REL_S_INT12/1 -> AND_S12/1
  REL_S_INT13/1 -> AND_S13/1
  REL_S_INT14/1 -> AND_S14/1
  REL_S_INT15/1 -> AND_S15/1
  REL_S_INT17/1 -> AND_S17/1
  REL_S_INT2/1 -> AND_S2/1
  REL_S_INT3/1 -> AND_S3/1
  REL_S_INT4/1 -> AND_S4/1
  REL_S_INT5/1 -> AND_S5/1
  REL_S_INT6/1 -> AND_S6/1
  REL_S_INT7/1 -> AND_S7/1
  REL_S_INT8/1 -> AND_S8/1
  REL_S_INT9/1 -> AND_S9/1
  SELECT_INT/1 -> REL_S_INT1/2, REL_S_INT2/2, REL_S_INT3/2, REL_S_INT4/2, REL_S_INT5/2, REL_S_INT6/2, REL_S_INT7/2, REL_S_INT8/2, REL_S_INT14/2, REL_S_INT15/2, REL_S_INT17/2, REL_S_INT13/2, REL_S_INT12/2, REL_S_INT11/2, REL_S_INT10/2, REL_S_INT9/2
  TIME1_NY/1 -> AND_S2/2
  TIME1_Y/1 -> AND_S1/2
  TIME2_NY/1 -> AND_S4/2
  TIME2_Y/1 -> AND_S3/2
  TIME3_NY/1 -> AND_S6/2
  TIME3_Y/1 -> AND_S5/2
  TIME4_NY/1 -> AND_S8/2
  TIME4_Y/1 -> AND_S7/2
  TIME5_NY/1 -> AND_S10/2
  TIME5_Y/1 -> AND_S9/2
  TIME6_NY/1 -> AND_S12/2
  TIME6_Y/1 -> AND_S11/2
  TIME7_NY/1 -> AND_S14/2
  TIME7_Y/1 -> AND_S13/2
  TIME8_NY/1 -> AND_S17/2
  TIME8_Y/1 -> AND_S15/2

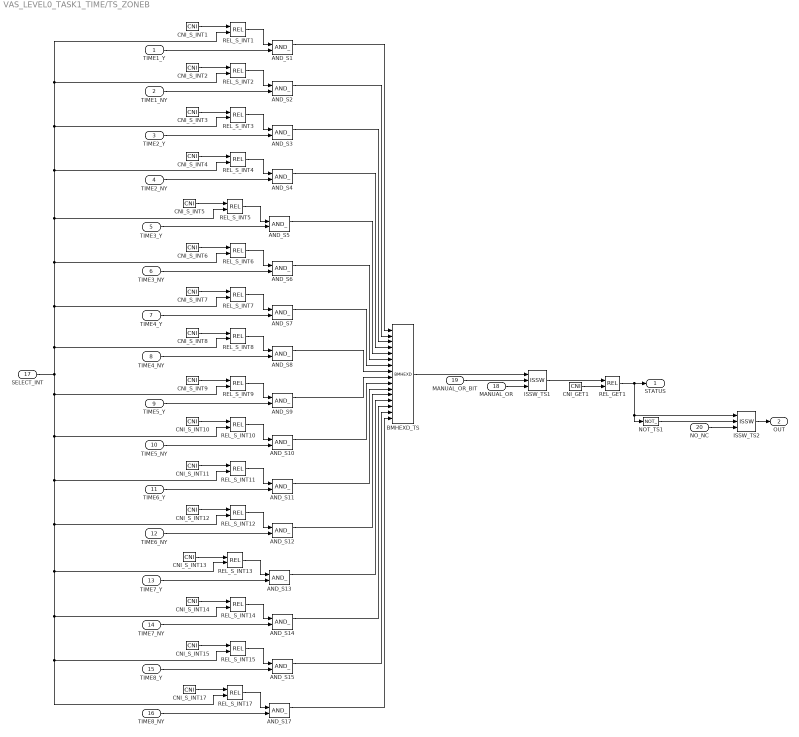
== system VAS_LEVEL0_TASK1_TIME/TS_ZONEB ==
  TIME1_Y : Inport  Port=1
  TIME1_NY : Inport  Port=2
  TIME2_Y : Inport  Port=3
  TIME2_NY : Inport  Port=4
  TIME3_Y : Inport  Port=5
  TIME3_NY : Inport  Port=6
  TIME4_Y : Inport  Port=7
  TIME4_NY : Inport  Port=8
  TIME5_Y : Inport  Port=9
  TIME5_NY : Inport  Port=10
  TIME6_Y : Inport  Port=11
  TIME6_NY : Inport  Port=12
  TIME7_Y : Inport  Port=13
  TIME7_NY : Inport  Port=14
  TIME8_Y : Inport  Port=15
  TIME8_NY : Inport  Port=16
  SELECT_INT : Inport  Port=17
  MANUAL_OR : Inport  Port=18
  MANUAL_OR_BIT : Inport  Port=19
  NO_NC : Inport  Port=20
  AND_S{1..15,17} (16 alike) : logiclib/AND_
  BMHEXD_TS : logiclib/BMHEXD  shift=0
  CNI_GET1 : mathlib/CNI  icn=1
  CNI_S_INT1 : mathlib/CNI  icn=0
  CNI_S_INT10 : mathlib/CNI  icn=9
  CNI_S_INT11 : mathlib/CNI  icn=10
  CNI_S_INT12 : mathlib/CNI  icn=11
  CNI_S_INT13 : mathlib/CNI  icn=12
  CNI_S_INT14 : mathlib/CNI  icn=13
  CNI_S_INT15 : mathlib/CNI  icn=14
  CNI_S_INT17 : mathlib/CNI  icn=15
  CNI_S_INT2 : mathlib/CNI  icn=1
  CNI_S_INT3 : mathlib/CNI  icn=2
  CNI_S_INT4 : mathlib/CNI  icn=3
  CNI_S_INT5 : mathlib/CNI  icn=4
  CNI_S_INT6 : mathlib/CNI  icn=5
  CNI_S_INT7 : mathlib/CNI  icn=6
  CNI_S_INT8 : mathlib/CNI  icn=7
  CNI_S_INT9 : mathlib/CNI  icn=8
  ISSW_TS1 : logiclib/ISSW
  ISSW_TS2 : logiclib/ISSW
  NOT_TS1 : logiclib/NOT_
  REL_GET1 : mathlib/REL  irel=6: greater or equal (>=)
  REL_S_INT{1..15,17} (16 alike) : mathlib/REL  irel=1: equality (==)
  STATUS : Outport  Port=1
  OUT : Outport  Port=2
  wires:
  AND_S1/1 -> BMHEXD_TS/1
  AND_S10/1 -> BMHEXD_TS/10
  AND_S11/1 -> BMHEXD_TS/11
  AND_S12/1 -> BMHEXD_TS/12
  AND_S13/1 -> BMHEXD_TS/13
  AND_S14/1 -> BMHEXD_TS/14
  AND_S15/1 -> BMHEXD_TS/15
  AND_S17/1 -> BMHEXD_TS/16
  AND_S2/1 -> BMHEXD_TS/2
  AND_S3/1 -> BMHEXD_TS/3
  AND_S4/1 -> BMHEXD_TS/4
  AND_S5/1 -> BMHEXD_TS/5
  AND_S6/1 -> BMHEXD_TS/6
  AND_S7/1 -> BMHEXD_TS/7
  AND_S8/1 -> BMHEXD_TS/8
  AND_S9/1 -> BMHEXD_TS/9
  BMHEXD_TS/1 -> ISSW_TS1/1
  CNI_GET1/1 -> REL_GET1/2
  CNI_S_INT1/1 -> REL_S_INT1/1
  CNI_S_INT10/1 -> REL_S_INT10/1
  CNI_S_INT11/1 -> REL_S_INT11/1
  CNI_S_INT12/1 -> REL_S_INT12/1
  CNI_S_INT13/1 -> REL_S_INT13/1
  CNI_S_INT14/1 -> REL_S_INT14/1
  CNI_S_INT15/1 -> REL_S_INT15/1
  CNI_S_INT17/1 -> REL_S_INT17/1
  CNI_S_INT2/1 -> REL_S_INT2/1
  CNI_S_INT3/1 -> REL_S_INT3/1
  CNI_S_INT4/1 -> REL_S_INT4/1
  CNI_S_INT5/1 -> REL_S_INT5/1
  CNI_S_INT6/1 -> REL_S_INT6/1
  CNI_S_INT7/1 -> REL_S_INT7/1
  CNI_S_INT8/1 -> REL_S_INT8/1
  CNI_S_INT9/1 -> REL_S_INT9/1
  ISSW_TS1/1 -> REL_GET1/1
  ISSW_TS2/1 -> OUT/1
  MANUAL_OR/1 -> ISSW_TS1/3
  MANUAL_OR_BIT/1 -> ISSW_TS1/2
  NOT_TS1/1 -> ISSW_TS2/2
  NO_NC/1 -> ISSW_TS2/3
  REL_GET1/1 -> STATUS/1, ISSW_TS2/1, NOT_TS1/1
  REL_S_INT1/1 -> AND_S1/1
  REL_S_INT10/1 -> AND_S10/1
  REL_S_INT11/1 -> AND_S11/1
  REL_S_INT12/1 -> AND_S12/1
  REL_S_INT13/1 -> AND_S13/1
  REL_S_INT14/1 -> AND_S14/1
  REL_S_INT15/1 -> AND_S15/1
  REL_S_INT17/1 -> AND_S17/1
  REL_S_INT2/1 -> AND_S2/1
  REL_S_INT3/1 -> AND_S3/1
  REL_S_INT4/1 -> AND_S4/1
  REL_S_INT5/1 -> AND_S5/1
  REL_S_INT6/1 -> AND_S6/1
  REL_S_INT7/1 -> AND_S7/1
  REL_S_INT8/1 -> AND_S8/1
  REL_S_INT9/1 -> AND_S9/1
  SELECT_INT/1 -> REL_S_INT1/2, REL_S_INT2/2, REL_S_INT3/2, REL_S_INT4/2, REL_S_INT5/2, REL_S_INT6/2, REL_S_INT7/2, REL_S_INT8/2, REL_S_INT14/2, REL_S_INT15/2, REL_S_INT17/2, REL_S_INT13/2, REL_S_INT12/2, REL_S_INT11/2, REL_S_INT10/2, REL_S_INT9/2
  TIME1_NY/1 -> AND_S2/2
  TIME1_Y/1 -> AND_S1/2
  TIME2_NY/1 -> AND_S4/2
  TIME2_Y/1 -> AND_S3/2
  TIME3_NY/1 -> AND_S6/2
  TIME3_Y/1 -> AND_S5/2
  TIME4_NY/1 -> AND_S8/2
  TIME4_Y/1 -> AND_S7/2
  TIME5_NY/1 -> AND_S10/2
  TIME5_Y/1 -> AND_S9/2
  TIME6_NY/1 -> AND_S12/2
  TIME6_Y/1 -> AND_S11/2
  TIME7_NY/1 -> AND_S14/2
  TIME7_Y/1 -> AND_S13/2
  TIME8_NY/1 -> AND_S17/2
  TIME8_Y/1 -> AND_S15/2

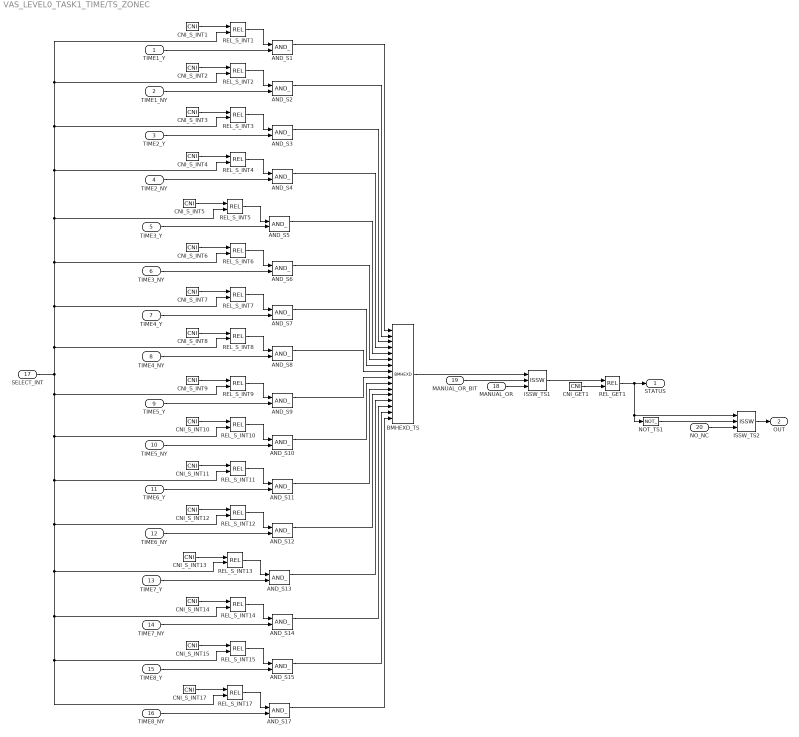
== system VAS_LEVEL0_TASK1_TIME/TS_ZONEC ==
  TIME1_Y : Inport  Port=1
  TIME1_NY : Inport  Port=2
  TIME2_Y : Inport  Port=3
  TIME2_NY : Inport  Port=4
  TIME3_Y : Inport  Port=5
  TIME3_NY : Inport  Port=6
  TIME4_Y : Inport  Port=7
  TIME4_NY : Inport  Port=8
  TIME5_Y : Inport  Port=9
  TIME5_NY : Inport  Port=10
  TIME6_Y : Inport  Port=11
  TIME6_NY : Inport  Port=12
  TIME7_Y : Inport  Port=13
  TIME7_NY : Inport  Port=14
  TIME8_Y : Inport  Port=15
  TIME8_NY : Inport  Port=16
  SELECT_INT : Inport  Port=17
  MANUAL_OR : Inport  Port=18
  MANUAL_OR_BIT : Inport  Port=19
  NO_NC : Inport  Port=20
  AND_S{1..15,17} (16 alike) : logiclib/AND_
  BMHEXD_TS : logiclib/BMHEXD  shift=0
  CNI_GET1 : mathlib/CNI  icn=1
  CNI_S_INT1 : mathlib/CNI  icn=0
  CNI_S_INT10 : mathlib/CNI  icn=9
  CNI_S_INT11 : mathlib/CNI  icn=10
  CNI_S_INT12 : mathlib/CNI  icn=11
  CNI_S_INT13 : mathlib/CNI  icn=12
  CNI_S_INT14 : mathlib/CNI  icn=13
  CNI_S_INT15 : mathlib/CNI  icn=14
  CNI_S_INT17 : mathlib/CNI  icn=15
  CNI_S_INT2 : mathlib/CNI  icn=1
  CNI_S_INT3 : mathlib/CNI  icn=2
  CNI_S_INT4 : mathlib/CNI  icn=3
  CNI_S_INT5 : mathlib/CNI  icn=4
  CNI_S_INT6 : mathlib/CNI  icn=5
  CNI_S_INT7 : mathlib/CNI  icn=6
  CNI_S_INT8 : mathlib/CNI  icn=7
  CNI_S_INT9 : mathlib/CNI  icn=8
  ISSW_TS1 : logiclib/ISSW
  ISSW_TS2 : logiclib/ISSW
  NOT_TS1 : logiclib/NOT_
  REL_GET1 : mathlib/REL  irel=6: greater or equal (>=)
  REL_S_INT{1..15,17} (16 alike) : mathlib/REL  irel=1: equality (==)
  STATUS : Outport  Port=1
  OUT : Outport  Port=2
  wires:
  AND_S1/1 -> BMHEXD_TS/1
  AND_S10/1 -> BMHEXD_TS/10
  AND_S11/1 -> BMHEXD_TS/11
  AND_S12/1 -> BMHEXD_TS/12
  AND_S13/1 -> BMHEXD_TS/13
  AND_S14/1 -> BMHEXD_TS/14
  AND_S15/1 -> BMHEXD_TS/15
  AND_S17/1 -> BMHEXD_TS/16
  AND_S2/1 -> BMHEXD_TS/2
  AND_S3/1 -> BMHEXD_TS/3
  AND_S4/1 -> BMHEXD_TS/4
  AND_S5/1 -> BMHEXD_TS/5
  AND_S6/1 -> BMHEXD_TS/6
  AND_S7/1 -> BMHEXD_TS/7
  AND_S8/1 -> BMHEXD_TS/8
  AND_S9/1 -> BMHEXD_TS/9
  BMHEXD_TS/1 -> ISSW_TS1/1
  CNI_GET1/1 -> REL_GET1/2
  CNI_S_INT1/1 -> REL_S_INT1/1
  CNI_S_INT10/1 -> REL_S_INT10/1
  CNI_S_INT11/1 -> REL_S_INT11/1
  CNI_S_INT12/1 -> REL_S_INT12/1
  CNI_S_INT13/1 -> REL_S_INT13/1
  CNI_S_INT14/1 -> REL_S_INT14/1
  CNI_S_INT15/1 -> REL_S_INT15/1
  CNI_S_INT17/1 -> REL_S_INT17/1
  CNI_S_INT2/1 -> REL_S_INT2/1
  CNI_S_INT3/1 -> REL_S_INT3/1
  CNI_S_INT4/1 -> REL_S_INT4/1
  CNI_S_INT5/1 -> REL_S_INT5/1
  CNI_S_INT6/1 -> REL_S_INT6/1
  CNI_S_INT7/1 -> REL_S_INT7/1
  CNI_S_INT8/1 -> REL_S_INT8/1
  CNI_S_INT9/1 -> REL_S_INT9/1
  ISSW_TS1/1 -> REL_GET1/1
  ISSW_TS2/1 -> OUT/1
  MANUAL_OR/1 -> ISSW_TS1/3
  MANUAL_OR_BIT/1 -> ISSW_TS1/2
  NOT_TS1/1 -> ISSW_TS2/2
  NO_NC/1 -> ISSW_TS2/3
  REL_GET1/1 -> STATUS/1, ISSW_TS2/1, NOT_TS1/1
  REL_S_INT1/1 -> AND_S1/1
  REL_S_INT10/1 -> AND_S10/1
  REL_S_INT11/1 -> AND_S11/1
  REL_S_INT12/1 -> AND_S12/1
  REL_S_INT13/1 -> AND_S13/1
  REL_S_INT14/1 -> AND_S14/1
  REL_S_INT15/1 -> AND_S15/1
  REL_S_INT17/1 -> AND_S17/1
  REL_S_INT2/1 -> AND_S2/1
  REL_S_INT3/1 -> AND_S3/1
  REL_S_INT4/1 -> AND_S4/1
  REL_S_INT5/1 -> AND_S5/1
  REL_S_INT6/1 -> AND_S6/1
  REL_S_INT7/1 -> AND_S7/1
  REL_S_INT8/1 -> AND_S8/1
  REL_S_INT9/1 -> AND_S9/1
  SELECT_INT/1 -> REL_S_INT1/2, REL_S_INT2/2, REL_S_INT3/2, REL_S_INT4/2, REL_S_INT5/2, REL_S_INT6/2, REL_S_INT7/2, REL_S_INT8/2, REL_S_INT14/2, REL_S_INT15/2, REL_S_INT17/2, REL_S_INT13/2, REL_S_INT12/2, REL_S_INT11/2, REL_S_INT10/2, REL_S_INT9/2
  TIME1_NY/1 -> AND_S2/2
  TIME1_Y/1 -> AND_S1/2
  TIME2_NY/1 -> AND_S4/2
  TIME2_Y/1 -> AND_S3/2
  TIME3_NY/1 -> AND_S6/2
  TIME3_Y/1 -> AND_S5/2
  TIME4_NY/1 -> AND_S8/2
  TIME4_Y/1 -> AND_S7/2
  TIME5_NY/1 -> AND_S10/2
  TIME5_Y/1 -> AND_S9/2
  TIME6_NY/1 -> AND_S12/2
  TIME6_Y/1 -> AND_S11/2
  TIME7_NY/1 -> AND_S14/2
  TIME7_Y/1 -> AND_S13/2
  TIME8_NY/1 -> AND_S17/2
  TIME8_Y/1 -> AND_S15/2

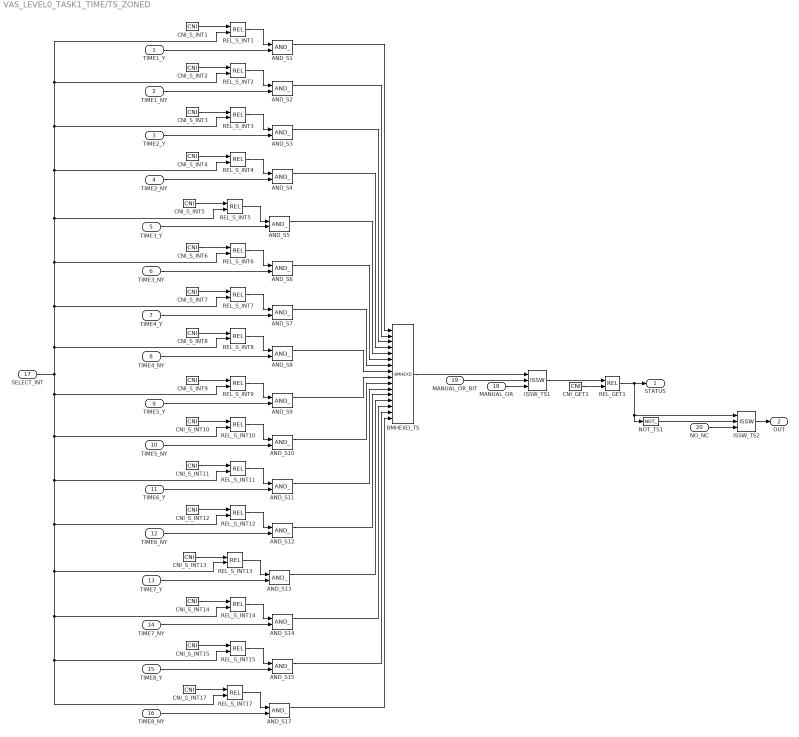
== system VAS_LEVEL0_TASK1_TIME/TS_ZONED ==
  TIME1_Y : Inport  Port=1
  TIME1_NY : Inport  Port=2
  TIME2_Y : Inport  Port=3
  TIME2_NY : Inport  Port=4
  TIME3_Y : Inport  Port=5
  TIME3_NY : Inport  Port=6
  TIME4_Y : Inport  Port=7
  TIME4_NY : Inport  Port=8
  TIME5_Y : Inport  Port=9
  TIME5_NY : Inport  Port=10
  TIME6_Y : Inport  Port=11
  TIME6_NY : Inport  Port=12
  TIME7_Y : Inport  Port=13
  TIME7_NY : Inport  Port=14
  TIME8_Y : Inport  Port=15
  TIME8_NY : Inport  Port=16
  SELECT_INT : Inport  Port=17
  MANUAL_OR : Inport  Port=18
  MANUAL_OR_BIT : Inport  Port=19
  NO_NC : Inport  Port=20
  AND_S{1..15,17} (16 alike) : logiclib/AND_
  BMHEXD_TS : logiclib/BMHEXD  shift=0
  CNI_GET1 : mathlib/CNI  icn=1
  CNI_S_INT1 : mathlib/CNI  icn=0
  CNI_S_INT10 : mathlib/CNI  icn=9
  CNI_S_INT11 : mathlib/CNI  icn=10
  CNI_S_INT12 : mathlib/CNI  icn=11
  CNI_S_INT13 : mathlib/CNI  icn=12
  CNI_S_INT14 : mathlib/CNI  icn=13
  CNI_S_INT15 : mathlib/CNI  icn=14
  CNI_S_INT17 : mathlib/CNI  icn=15
  CNI_S_INT2 : mathlib/CNI  icn=1
  CNI_S_INT3 : mathlib/CNI  icn=2
  CNI_S_INT4 : mathlib/CNI  icn=3
  CNI_S_INT5 : mathlib/CNI  icn=4
  CNI_S_INT6 : mathlib/CNI  icn=5
  CNI_S_INT7 : mathlib/CNI  icn=6
  CNI_S_INT8 : mathlib/CNI  icn=7
  CNI_S_INT9 : mathlib/CNI  icn=8
  ISSW_TS1 : logiclib/ISSW
  ISSW_TS2 : logiclib/ISSW
  NOT_TS1 : logiclib/NOT_
  REL_GET1 : mathlib/REL  irel=6: greater or equal (>=)
  REL_S_INT{1..15,17} (16 alike) : mathlib/REL  irel=1: equality (==)
  STATUS : Outport  Port=1
  OUT : Outport  Port=2
  wires:
  AND_S1/1 -> BMHEXD_TS/1
  AND_S10/1 -> BMHEXD_TS/10
  AND_S11/1 -> BMHEXD_TS/11
  AND_S12/1 -> BMHEXD_TS/12
  AND_S13/1 -> BMHEXD_TS/13
  AND_S14/1 -> BMHEXD_TS/14
  AND_S15/1 -> BMHEXD_TS/15
  AND_S17/1 -> BMHEXD_TS/16
  AND_S2/1 -> BMHEXD_TS/2
  AND_S3/1 -> BMHEXD_TS/3
  AND_S4/1 -> BMHEXD_TS/4
  AND_S5/1 -> BMHEXD_TS/5
  AND_S6/1 -> BMHEXD_TS/6
  AND_S7/1 -> BMHEXD_TS/7
  AND_S8/1 -> BMHEXD_TS/8
  AND_S9/1 -> BMHEXD_TS/9
  BMHEXD_TS/1 -> ISSW_TS1/1
  CNI_GET1/1 -> REL_GET1/2
  CNI_S_INT1/1 -> REL_S_INT1/1
  CNI_S_INT10/1 -> REL_S_INT10/1
  CNI_S_INT11/1 -> REL_S_INT11/1
  CNI_S_INT12/1 -> REL_S_INT12/1
  CNI_S_INT13/1 -> REL_S_INT13/1
  CNI_S_INT14/1 -> REL_S_INT14/1
  CNI_S_INT15/1 -> REL_S_INT15/1
  CNI_S_INT17/1 -> REL_S_INT17/1
  CNI_S_INT2/1 -> REL_S_INT2/1
  CNI_S_INT3/1 -> REL_S_INT3/1
  CNI_S_INT4/1 -> REL_S_INT4/1
  CNI_S_INT5/1 -> REL_S_INT5/1
  CNI_S_INT6/1 -> REL_S_INT6/1
  CNI_S_INT7/1 -> REL_S_INT7/1
  CNI_S_INT8/1 -> REL_S_INT8/1
  CNI_S_INT9/1 -> REL_S_INT9/1
  ISSW_TS1/1 -> REL_GET1/1
  ISSW_TS2/1 -> OUT/1
  MANUAL_OR/1 -> ISSW_TS1/3
  MANUAL_OR_BIT/1 -> ISSW_TS1/2
  NOT_TS1/1 -> ISSW_TS2/2
  NO_NC/1 -> ISSW_TS2/3
  REL_GET1/1 -> STATUS/1, ISSW_TS2/1, NOT_TS1/1
  REL_S_INT1/1 -> AND_S1/1
  REL_S_INT10/1 -> AND_S10/1
  REL_S_INT11/1 -> AND_S11/1
  REL_S_INT12/1 -> AND_S12/1
  REL_S_INT13/1 -> AND_S13/1
  REL_S_INT14/1 -> AND_S14/1
  REL_S_INT15/1 -> AND_S15/1
  REL_S_INT17/1 -> AND_S17/1
  REL_S_INT2/1 -> AND_S2/1
  REL_S_INT3/1 -> AND_S3/1
  REL_S_INT4/1 -> AND_S4/1
  REL_S_INT5/1 -> AND_S5/1
  REL_S_INT6/1 -> AND_S6/1
  REL_S_INT7/1 -> AND_S7/1
  REL_S_INT8/1 -> AND_S8/1
  REL_S_INT9/1 -> AND_S9/1
  SELECT_INT/1 -> REL_S_INT1/2, REL_S_INT2/2, REL_S_INT3/2, REL_S_INT4/2, REL_S_INT5/2, REL_S_INT6/2, REL_S_INT7/2, REL_S_INT8/2, REL_S_INT14/2, REL_S_INT15/2, REL_S_INT17/2, REL_S_INT13/2, REL_S_INT12/2, REL_S_INT11/2, REL_S_INT10/2, REL_S_INT9/2
  TIME1_NY/1 -> AND_S2/2
  TIME1_Y/1 -> AND_S1/2
  TIME2_NY/1 -> AND_S4/2
  TIME2_Y/1 -> AND_S3/2
  TIME3_NY/1 -> AND_S6/2
  TIME3_Y/1 -> AND_S5/2
  TIME4_NY/1 -> AND_S8/2
  TIME4_Y/1 -> AND_S7/2
  TIME5_NY/1 -> AND_S10/2
  TIME5_Y/1 -> AND_S9/2
  TIME6_NY/1 -> AND_S12/2
  TIME6_Y/1 -> AND_S11/2
  TIME7_NY/1 -> AND_S14/2
  TIME7_Y/1 -> AND_S13/2
  TIME8_NY/1 -> AND_S17/2
  TIME8_Y/1 -> AND_S15/2

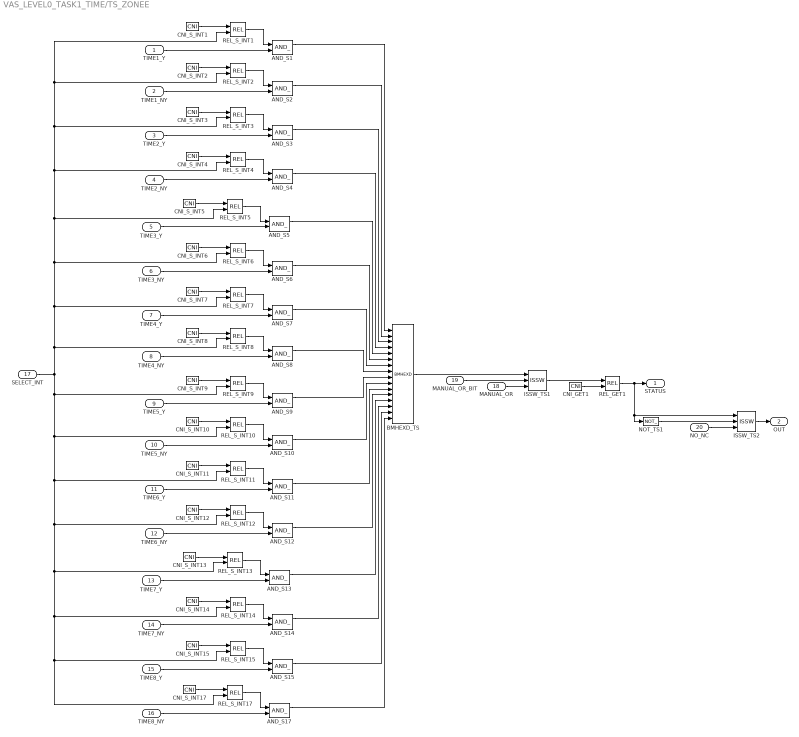
== system VAS_LEVEL0_TASK1_TIME/TS_ZONEE ==
  TIME1_Y : Inport  Port=1
  TIME1_NY : Inport  Port=2
  TIME2_Y : Inport  Port=3
  TIME2_NY : Inport  Port=4
  TIME3_Y : Inport  Port=5
  TIME3_NY : Inport  Port=6
  TIME4_Y : Inport  Port=7
  TIME4_NY : Inport  Port=8
  TIME5_Y : Inport  Port=9
  TIME5_NY : Inport  Port=10
  TIME6_Y : Inport  Port=11
  TIME6_NY : Inport  Port=12
  TIME7_Y : Inport  Port=13
  TIME7_NY : Inport  Port=14
  TIME8_Y : Inport  Port=15
  TIME8_NY : Inport  Port=16
  SELECT_INT : Inport  Port=17
  MANUAL_OR : Inport  Port=18
  MANUAL_OR_BIT : Inport  Port=19
  NO_NC : Inport  Port=20
  AND_S{1..15,17} (16 alike) : logiclib/AND_
  BMHEXD_TS : logiclib/BMHEXD  shift=0
  CNI_GET1 : mathlib/CNI  icn=1
  CNI_S_INT1 : mathlib/CNI  icn=0
  CNI_S_INT10 : mathlib/CNI  icn=9
  CNI_S_INT11 : mathlib/CNI  icn=10
  CNI_S_INT12 : mathlib/CNI  icn=11
  CNI_S_INT13 : mathlib/CNI  icn=12
  CNI_S_INT14 : mathlib/CNI  icn=13
  CNI_S_INT15 : mathlib/CNI  icn=14
  CNI_S_INT17 : mathlib/CNI  icn=15
  CNI_S_INT2 : mathlib/CNI  icn=1
  CNI_S_INT3 : mathlib/CNI  icn=2
  CNI_S_INT4 : mathlib/CNI  icn=3
  CNI_S_INT5 : mathlib/CNI  icn=4
  CNI_S_INT6 : mathlib/CNI  icn=5
  CNI_S_INT7 : mathlib/CNI  icn=6
  CNI_S_INT8 : mathlib/CNI  icn=7
  CNI_S_INT9 : mathlib/CNI  icn=8
  ISSW_TS1 : logiclib/ISSW
  ISSW_TS2 : logiclib/ISSW
  NOT_TS1 : logiclib/NOT_
  REL_GET1 : mathlib/REL  irel=6: greater or equal (>=)
  REL_S_INT{1..15,17} (16 alike) : mathlib/REL  irel=1: equality (==)
  STATUS : Outport  Port=1
  OUT : Outport  Port=2
  wires:
  AND_S1/1 -> BMHEXD_TS/1
  AND_S10/1 -> BMHEXD_TS/10
  AND_S11/1 -> BMHEXD_TS/11
  AND_S12/1 -> BMHEXD_TS/12
  AND_S13/1 -> BMHEXD_TS/13
  AND_S14/1 -> BMHEXD_TS/14
  AND_S15/1 -> BMHEXD_TS/15
  AND_S17/1 -> BMHEXD_TS/16
  AND_S2/1 -> BMHEXD_TS/2
  AND_S3/1 -> BMHEXD_TS/3
  AND_S4/1 -> BMHEXD_TS/4
  AND_S5/1 -> BMHEXD_TS/5
  AND_S6/1 -> BMHEXD_TS/6
  AND_S7/1 -> BMHEXD_TS/7
  AND_S8/1 -> BMHEXD_TS/8
  AND_S9/1 -> BMHEXD_TS/9
  BMHEXD_TS/1 -> ISSW_TS1/1
  CNI_GET1/1 -> REL_GET1/2
  CNI_S_INT1/1 -> REL_S_INT1/1
  CNI_S_INT10/1 -> REL_S_INT10/1
  CNI_S_INT11/1 -> REL_S_INT11/1
  CNI_S_INT12/1 -> REL_S_INT12/1
  CNI_S_INT13/1 -> REL_S_INT13/1
  CNI_S_INT14/1 -> REL_S_INT14/1
  CNI_S_INT15/1 -> REL_S_INT15/1
  CNI_S_INT17/1 -> REL_S_INT17/1
  CNI_S_INT2/1 -> REL_S_INT2/1
  CNI_S_INT3/1 -> REL_S_INT3/1
  CNI_S_INT4/1 -> REL_S_INT4/1
  CNI_S_INT5/1 -> REL_S_INT5/1
  CNI_S_INT6/1 -> REL_S_INT6/1
  CNI_S_INT7/1 -> REL_S_INT7/1
  CNI_S_INT8/1 -> REL_S_INT8/1
  CNI_S_INT9/1 -> REL_S_INT9/1
  ISSW_TS1/1 -> REL_GET1/1
  ISSW_TS2/1 -> OUT/1
  MANUAL_OR/1 -> ISSW_TS1/3
  MANUAL_OR_BIT/1 -> ISSW_TS1/2
  NOT_TS1/1 -> ISSW_TS2/2
  NO_NC/1 -> ISSW_TS2/3
  REL_GET1/1 -> STATUS/1, ISSW_TS2/1, NOT_TS1/1
  REL_S_INT1/1 -> AND_S1/1
  REL_S_INT10/1 -> AND_S10/1
  REL_S_INT11/1 -> AND_S11/1
  REL_S_INT12/1 -> AND_S12/1
  REL_S_INT13/1 -> AND_S13/1
  REL_S_INT14/1 -> AND_S14/1
  REL_S_INT15/1 -> AND_S15/1
  REL_S_INT17/1 -> AND_S17/1
  REL_S_INT2/1 -> AND_S2/1
  REL_S_INT3/1 -> AND_S3/1
  REL_S_INT4/1 -> AND_S4/1
  REL_S_INT5/1 -> AND_S5/1
  REL_S_INT6/1 -> AND_S6/1
  REL_S_INT7/1 -> AND_S7/1
  REL_S_INT8/1 -> AND_S8/1
  REL_S_INT9/1 -> AND_S9/1
  SELECT_INT/1 -> REL_S_INT1/2, REL_S_INT2/2, REL_S_INT3/2, REL_S_INT4/2, REL_S_INT5/2, REL_S_INT6/2, REL_S_INT7/2, REL_S_INT8/2, REL_S_INT14/2, REL_S_INT15/2, REL_S_INT17/2, REL_S_INT13/2, REL_S_INT12/2, REL_S_INT11/2, REL_S_INT10/2, REL_S_INT9/2
  TIME1_NY/1 -> AND_S2/2
  TIME1_Y/1 -> AND_S1/2
  TIME2_NY/1 -> AND_S4/2
  TIME2_Y/1 -> AND_S3/2
  TIME3_NY/1 -> AND_S6/2
  TIME3_Y/1 -> AND_S5/2
  TIME4_NY/1 -> AND_S8/2
  TIME4_Y/1 -> AND_S7/2
  TIME5_NY/1 -> AND_S10/2
  TIME5_Y/1 -> AND_S9/2
  TIME6_NY/1 -> AND_S12/2
  TIME6_Y/1 -> AND_S11/2
  TIME7_NY/1 -> AND_S14/2
  TIME7_Y/1 -> AND_S13/2
  TIME8_NY/1 -> AND_S17/2
  TIME8_Y/1 -> AND_S15/2

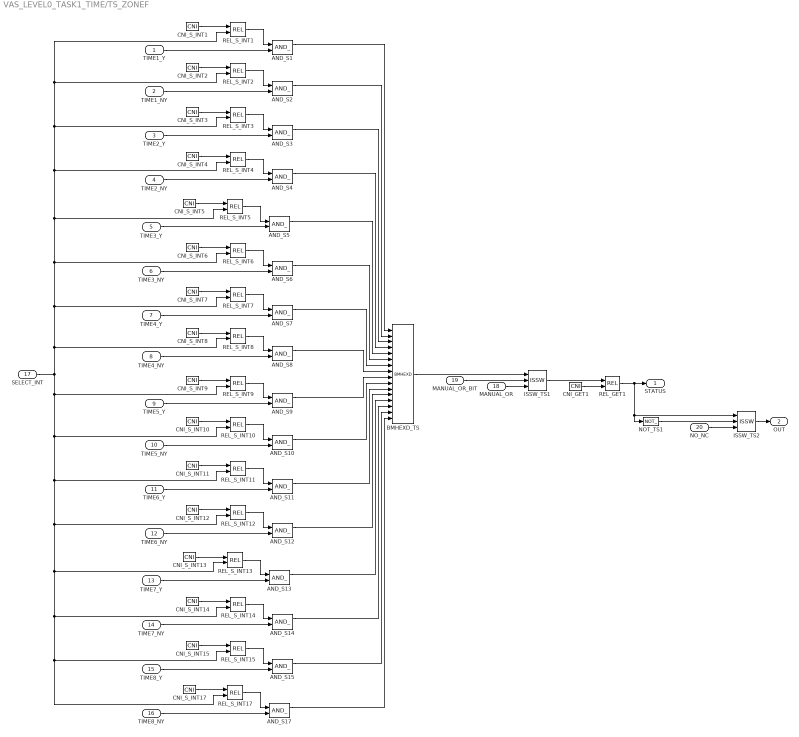
== system VAS_LEVEL0_TASK1_TIME/TS_ZONEF ==
  TIME1_Y : Inport  Port=1
  TIME1_NY : Inport  Port=2
  TIME2_Y : Inport  Port=3
  TIME2_NY : Inport  Port=4
  TIME3_Y : Inport  Port=5
  TIME3_NY : Inport  Port=6
  TIME4_Y : Inport  Port=7
  TIME4_NY : Inport  Port=8
  TIME5_Y : Inport  Port=9
  TIME5_NY : Inport  Port=10
  TIME6_Y : Inport  Port=11
  TIME6_NY : Inport  Port=12
  TIME7_Y : Inport  Port=13
  TIME7_NY : Inport  Port=14
  TIME8_Y : Inport  Port=15
  TIME8_NY : Inport  Port=16
  SELECT_INT : Inport  Port=17
  MANUAL_OR : Inport  Port=18
  MANUAL_OR_BIT : Inport  Port=19
  NO_NC : Inport  Port=20
  AND_S{1..15,17} (16 alike) : logiclib/AND_
  BMHEXD_TS : logiclib/BMHEXD  shift=0
  CNI_GET1 : mathlib/CNI  icn=1
  CNI_S_INT1 : mathlib/CNI  icn=0
  CNI_S_INT10 : mathlib/CNI  icn=9
  CNI_S_INT11 : mathlib/CNI  icn=10
  CNI_S_INT12 : mathlib/CNI  icn=11
  CNI_S_INT13 : mathlib/CNI  icn=12
  CNI_S_INT14 : mathlib/CNI  icn=13
  CNI_S_INT15 : mathlib/CNI  icn=14
  CNI_S_INT17 : mathlib/CNI  icn=15
  CNI_S_INT2 : mathlib/CNI  icn=1
  CNI_S_INT3 : mathlib/CNI  icn=2
  CNI_S_INT4 : mathlib/CNI  icn=3
  CNI_S_INT5 : mathlib/CNI  icn=4
  CNI_S_INT6 : mathlib/CNI  icn=5
  CNI_S_INT7 : mathlib/CNI  icn=6
  CNI_S_INT8 : mathlib/CNI  icn=7
  CNI_S_INT9 : mathlib/CNI  icn=8
  ISSW_TS1 : logiclib/ISSW
  ISSW_TS2 : logiclib/ISSW
  NOT_TS1 : logiclib/NOT_
  REL_GET1 : mathlib/REL  irel=6: greater or equal (>=)
  REL_S_INT{1..15,17} (16 alike) : mathlib/REL  irel=1: equality (==)
  STATUS : Outport  Port=1
  OUT : Outport  Port=2
  wires:
  AND_S1/1 -> BMHEXD_TS/1
  AND_S10/1 -> BMHEXD_TS/10
  AND_S11/1 -> BMHEXD_TS/11
  AND_S12/1 -> BMHEXD_TS/12
  AND_S13/1 -> BMHEXD_TS/13
  AND_S14/1 -> BMHEXD_TS/14
  AND_S15/1 -> BMHEXD_TS/15
  AND_S17/1 -> BMHEXD_TS/16
  AND_S2/1 -> BMHEXD_TS/2
  AND_S3/1 -> BMHEXD_TS/3
  AND_S4/1 -> BMHEXD_TS/4
  AND_S5/1 -> BMHEXD_TS/5
  AND_S6/1 -> BMHEXD_TS/6
  AND_S7/1 -> BMHEXD_TS/7
  AND_S8/1 -> BMHEXD_TS/8
  AND_S9/1 -> BMHEXD_TS/9
  BMHEXD_TS/1 -> ISSW_TS1/1
  CNI_GET1/1 -> REL_GET1/2
  CNI_S_INT1/1 -> REL_S_INT1/1
  CNI_S_INT10/1 -> REL_S_INT10/1
  CNI_S_INT11/1 -> REL_S_INT11/1
  CNI_S_INT12/1 -> REL_S_INT12/1
  CNI_S_INT13/1 -> REL_S_INT13/1
  CNI_S_INT14/1 -> REL_S_INT14/1
  CNI_S_INT15/1 -> REL_S_INT15/1
  CNI_S_INT17/1 -> REL_S_INT17/1
  CNI_S_INT2/1 -> REL_S_INT2/1
  CNI_S_INT3/1 -> REL_S_INT3/1
  CNI_S_INT4/1 -> REL_S_INT4/1
  CNI_S_INT5/1 -> REL_S_INT5/1
  CNI_S_INT6/1 -> REL_S_INT6/1
  CNI_S_INT7/1 -> REL_S_INT7/1
  CNI_S_INT8/1 -> REL_S_INT8/1
  CNI_S_INT9/1 -> REL_S_INT9/1
  ISSW_TS1/1 -> REL_GET1/1
  ISSW_TS2/1 -> OUT/1
  MANUAL_OR/1 -> ISSW_TS1/3
  MANUAL_OR_BIT/1 -> ISSW_TS1/2
  NOT_TS1/1 -> ISSW_TS2/2
  NO_NC/1 -> ISSW_TS2/3
  REL_GET1/1 -> STATUS/1, ISSW_TS2/1, NOT_TS1/1
  REL_S_INT1/1 -> AND_S1/1
  REL_S_INT10/1 -> AND_S10/1
  REL_S_INT11/1 -> AND_S11/1
  REL_S_INT12/1 -> AND_S12/1
  REL_S_INT13/1 -> AND_S13/1
  REL_S_INT14/1 -> AND_S14/1
  REL_S_INT15/1 -> AND_S15/1
  REL_S_INT17/1 -> AND_S17/1
  REL_S_INT2/1 -> AND_S2/1
  REL_S_INT3/1 -> AND_S3/1
  REL_S_INT4/1 -> AND_S4/1
  REL_S_INT5/1 -> AND_S5/1
  REL_S_INT6/1 -> AND_S6/1
  REL_S_INT7/1 -> AND_S7/1
  REL_S_INT8/1 -> AND_S8/1
  REL_S_INT9/1 -> AND_S9/1
  SELECT_INT/1 -> REL_S_INT1/2, REL_S_INT2/2, REL_S_INT3/2, REL_S_INT4/2, REL_S_INT5/2, REL_S_INT6/2, REL_S_INT7/2, REL_S_INT8/2, REL_S_INT14/2, REL_S_INT15/2, REL_S_INT17/2, REL_S_INT13/2, REL_S_INT12/2, REL_S_INT11/2, REL_S_INT10/2, REL_S_INT9/2
  TIME1_NY/1 -> AND_S2/2
  TIME1_Y/1 -> AND_S1/2
  TIME2_NY/1 -> AND_S4/2
  TIME2_Y/1 -> AND_S3/2
  TIME3_NY/1 -> AND_S6/2
  TIME3_Y/1 -> AND_S5/2
  TIME4_NY/1 -> AND_S8/2
  TIME4_Y/1 -> AND_S7/2
  TIME5_NY/1 -> AND_S10/2
  TIME5_Y/1 -> AND_S9/2
  TIME6_NY/1 -> AND_S12/2
  TIME6_Y/1 -> AND_S11/2
  TIME7_NY/1 -> AND_S14/2
  TIME7_Y/1 -> AND_S13/2
  TIME8_NY/1 -> AND_S17/2
  TIME8_Y/1 -> AND_S15/2

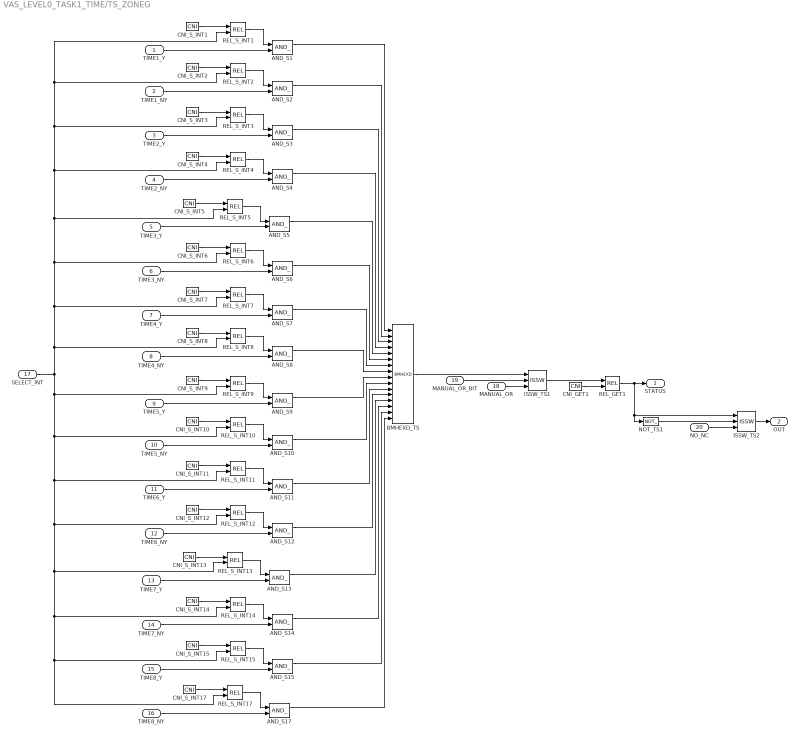
== system VAS_LEVEL0_TASK1_TIME/TS_ZONEG ==
  TIME1_Y : Inport  Port=1
  TIME1_NY : Inport  Port=2
  TIME2_Y : Inport  Port=3
  TIME2_NY : Inport  Port=4
  TIME3_Y : Inport  Port=5
  TIME3_NY : Inport  Port=6
  TIME4_Y : Inport  Port=7
  TIME4_NY : Inport  Port=8
  TIME5_Y : Inport  Port=9
  TIME5_NY : Inport  Port=10
  TIME6_Y : Inport  Port=11
  TIME6_NY : Inport  Port=12
  TIME7_Y : Inport  Port=13
  TIME7_NY : Inport  Port=14
  TIME8_Y : Inport  Port=15
  TIME8_NY : Inport  Port=16
  SELECT_INT : Inport  Port=17
  MANUAL_OR : Inport  Port=18
  MANUAL_OR_BIT : Inport  Port=19
  NO_NC : Inport  Port=20
  AND_S{1..15,17} (16 alike) : logiclib/AND_
  BMHEXD_TS : logiclib/BMHEXD  shift=0
  CNI_GET1 : mathlib/CNI  icn=1
  CNI_S_INT1 : mathlib/CNI  icn=0
  CNI_S_INT10 : mathlib/CNI  icn=9
  CNI_S_INT11 : mathlib/CNI  icn=10
  CNI_S_INT12 : mathlib/CNI  icn=11
  CNI_S_INT13 : mathlib/CNI  icn=12
  CNI_S_INT14 : mathlib/CNI  icn=13
  CNI_S_INT15 : mathlib/CNI  icn=14
  CNI_S_INT17 : mathlib/CNI  icn=15
  CNI_S_INT2 : mathlib/CNI  icn=1
  CNI_S_INT3 : mathlib/CNI  icn=2
  CNI_S_INT4 : mathlib/CNI  icn=3
  CNI_S_INT5 : mathlib/CNI  icn=4
  CNI_S_INT6 : mathlib/CNI  icn=5
  CNI_S_INT7 : mathlib/CNI  icn=6
  CNI_S_INT8 : mathlib/CNI  icn=7
  CNI_S_INT9 : mathlib/CNI  icn=8
  ISSW_TS1 : logiclib/ISSW
  ISSW_TS2 : logiclib/ISSW
  NOT_TS1 : logiclib/NOT_
  REL_GET1 : mathlib/REL  irel=6: greater or equal (>=)
  REL_S_INT{1..15,17} (16 alike) : mathlib/REL  irel=1: equality (==)
  STATUS : Outport  Port=1
  OUT : Outport  Port=2
  wires:
  AND_S1/1 -> BMHEXD_TS/1
  AND_S10/1 -> BMHEXD_TS/10
  AND_S11/1 -> BMHEXD_TS/11
  AND_S12/1 -> BMHEXD_TS/12
  AND_S13/1 -> BMHEXD_TS/13
  AND_S14/1 -> BMHEXD_TS/14
  AND_S15/1 -> BMHEXD_TS/15
  AND_S17/1 -> BMHEXD_TS/16
  AND_S2/1 -> BMHEXD_TS/2
  AND_S3/1 -> BMHEXD_TS/3
  AND_S4/1 -> BMHEXD_TS/4
  AND_S5/1 -> BMHEXD_TS/5
  AND_S6/1 -> BMHEXD_TS/6
  AND_S7/1 -> BMHEXD_TS/7
  AND_S8/1 -> BMHEXD_TS/8
  AND_S9/1 -> BMHEXD_TS/9
  BMHEXD_TS/1 -> ISSW_TS1/1
  CNI_GET1/1 -> REL_GET1/2
  CNI_S_INT1/1 -> REL_S_INT1/1
  CNI_S_INT10/1 -> REL_S_INT10/1
  CNI_S_INT11/1 -> REL_S_INT11/1
  CNI_S_INT12/1 -> REL_S_INT12/1
  CNI_S_INT13/1 -> REL_S_INT13/1
  CNI_S_INT14/1 -> REL_S_INT14/1
  CNI_S_INT15/1 -> REL_S_INT15/1
  CNI_S_INT17/1 -> REL_S_INT17/1
  CNI_S_INT2/1 -> REL_S_INT2/1
  CNI_S_INT3/1 -> REL_S_INT3/1
  CNI_S_INT4/1 -> REL_S_INT4/1
  CNI_S_INT5/1 -> REL_S_INT5/1
  CNI_S_INT6/1 -> REL_S_INT6/1
  CNI_S_INT7/1 -> REL_S_INT7/1
  CNI_S_INT8/1 -> REL_S_INT8/1
  CNI_S_INT9/1 -> REL_S_INT9/1
  ISSW_TS1/1 -> REL_GET1/1
  ISSW_TS2/1 -> OUT/1
  MANUAL_OR/1 -> ISSW_TS1/3
  MANUAL_OR_BIT/1 -> ISSW_TS1/2
  NOT_TS1/1 -> ISSW_TS2/2
  NO_NC/1 -> ISSW_TS2/3
  REL_GET1/1 -> STATUS/1, ISSW_TS2/1, NOT_TS1/1
  REL_S_INT1/1 -> AND_S1/1
  REL_S_INT10/1 -> AND_S10/1
  REL_S_INT11/1 -> AND_S11/1
  REL_S_INT12/1 -> AND_S12/1
  REL_S_INT13/1 -> AND_S13/1
  REL_S_INT14/1 -> AND_S14/1
  REL_S_INT15/1 -> AND_S15/1
  REL_S_INT17/1 -> AND_S17/1
  REL_S_INT2/1 -> AND_S2/1
  REL_S_INT3/1 -> AND_S3/1
  REL_S_INT4/1 -> AND_S4/1
  REL_S_INT5/1 -> AND_S5/1
  REL_S_INT6/1 -> AND_S6/1
  REL_S_INT7/1 -> AND_S7/1
  REL_S_INT8/1 -> AND_S8/1
  REL_S_INT9/1 -> AND_S9/1
  SELECT_INT/1 -> REL_S_INT1/2, REL_S_INT2/2, REL_S_INT3/2, REL_S_INT4/2, REL_S_INT5/2, REL_S_INT6/2, REL_S_INT7/2, REL_S_INT8/2, REL_S_INT14/2, REL_S_INT15/2, REL_S_INT17/2, REL_S_INT13/2, REL_S_INT12/2, REL_S_INT11/2, REL_S_INT10/2, REL_S_INT9/2
  TIME1_NY/1 -> AND_S2/2
  TIME1_Y/1 -> AND_S1/2
  TIME2_NY/1 -> AND_S4/2
  TIME2_Y/1 -> AND_S3/2
  TIME3_NY/1 -> AND_S6/2
  TIME3_Y/1 -> AND_S5/2
  TIME4_NY/1 -> AND_S8/2
  TIME4_Y/1 -> AND_S7/2
  TIME5_NY/1 -> AND_S10/2
  TIME5_Y/1 -> AND_S9/2
  TIME6_NY/1 -> AND_S12/2
  TIME6_Y/1 -> AND_S11/2
  TIME7_NY/1 -> AND_S14/2
  TIME7_Y/1 -> AND_S13/2
  TIME8_NY/1 -> AND_S17/2
  TIME8_Y/1 -> AND_S15/2
